simulink model "Drone_Response_v5"  (R2024b)
settings: Solver=VariableStepAuto  StartTime=0.0  StopTime=17.980265000000003  MaxStep=0.01  RelTol=1e-6  AbsTol=1e-8
model workspace (MAT data in the model file):
  Fx_gust = 1
  Fy_gust = 1
  Fz_gust = 0.5
  Ixx = 0.05
  Iyy = 0.05
  Izz = 0.1
  Kd_phi = 0.5
  Kd_psi = 0.12
  Kd_theta = 0.28
  Kd_x = 0.5
  Kd_y = 0.5
  Kd_z = 12
  Ki_phi = 0
  Ki_psi = 0
  Ki_theta = 0.28
  Ki_x = 0
  Ki_y = 0
  Ki_z = 0.1
  Kp_phi = 1
  Kp_psi = 0.012
  Kp_theta = 0.8
  Kp_x = 0.1
  Kp_y = 0.1
  Kp_z = 12
  N_phi = 100
  N_psi = 100
  N_theta = 100
  N_x = 100
  N_y = 100
  N_z = 100
  Tmax = 22.4649
  Tmin = 0
  d = 0.2
  disturbances_enabled = 0
  flight_mode = 3
  frozen_configuration.Name = "V3_conditioned_start"
  frozen_configuration.Kp = 0.753283912428
  frozen_configuration.Kd = 1.41064730788
  frozen_configuration.FeedforwardGain = 0.856563645814
  frozen_configuration.KpX = 0.1
  frozen_configuration.KdX = 0.192
  frozen_configuration.KpY = 0.1
  frozen_configuration.KdY = 0.192
  frozen_configuration.KpYaw = 0.012
  frozen_configuration.KdYaw = 0.12
  frozen_configuration.DragRate = 0
  frozen_configuration.ConditionAllFilters = 1
  frozen_configuration.Ki = 0.0024123505433
  frozen_filter_init_184 = 0.000968325935072
  frozen_filter_init_244 = -0.00996407378017
  frozen_filter_init_247 = 0.0189310533866
  frozen_filter_init_63 = 0.120731046274
  frozen_filter_init_8 = -0.00230151225217
  frozen_filter_init_92 = -0.00686694318858
  g = 9.81
  inv_m = 0.333333333333
  kf = 4e-05
  km = 1e-06
  m = 3
  mg = 29.43
  omega_hover = 399.217985567
  omega_init = 428.879353665
  phi0 = 0.0109224523708
  phi_des = 0
  phi_dot0 = -0.0602280499979
  phi_manual = 0
  pitch_pair_allocation = 2.5
  psi0 = 2.78260847334
  psi_des = 0
  psi_dot0 = 0.0811475700195
  psi_hold = 0
  psi_manual = 0
  rad_to_deg = 57.2957795131
  replay_collective_to_pair_thrust_N = 58
  replay_enabled = 1
  replay_hover_collective = 0.24829455053
  replay_hover_pair_thrust_scale_N = 51.3503013771
  response_axis_nx = -0.0174524064373
  response_axis_ny = 0
  response_axis_nz = 0.999847695156
  response_experiment_status = 'Frozen experimental replay: ascent training8.7805; reserved descent2.6653; full airborne0. NOT a general8/10 release.'
  response_manual_enable = timeseries
  response_manual_enable.Name = 'unnamed'
  response_manual_enable.DataInfo = tsdata.datametadata
  response_manual_enable.DataInfo.Interpolation = tsdata.interpolation
  response_manual_enable.DataInfo.Interpolation.Fhandle : function handle (value not decoded)
  response_manual_enable.DataInfo.Interpolation.Name = 'zoh'
  response_manual_enable.TimeInfo = tsdata.timemetadata
  response_manual_enable.TimeInfo.Length = 3
  response_manual_enable.TimeInfo.DuplicateTimes = 0
  response_manual_enable.TimeInfo.Time_ = [0; 5.880394; 17.980265]
  response_manual_enable.TimeInfo.Initialized = 1
  response_manual_enable.QualityInfo = tsdata.qualmetadata
  response_manual_enable.Data_ = [1; 0; 0]
  response_v5_status = 'Experimental controller design; general8/10 not achieved; manufacturer cap provisional'
  response_vertical_drag_rate = 0.5
  roll_motor_allocation = 1.25
  rtl_accel_ff_gain = 0.856563645814
  rtl_altitude_accel_command = timeseries
  rtl_altitude_accel_command.Name = 'unnamed'
  rtl_altitude_accel_command.DataInfo = tsdata.datametadata
  rtl_altitude_accel_command.DataInfo.Interpolation = tsdata.interpolation
  rtl_altitude_accel_command.DataInfo.Interpolation.Fhandle : function handle (value not decoded)
  rtl_altitude_accel_command.DataInfo.Interpolation.Name = 'linear'
  rtl_altitude_accel_command.TimeInfo = tsdata.timemetadata
  rtl_altitude_accel_command.TimeInfo.Length = 123
  rtl_altitude_accel_command.TimeInfo.DuplicateTimes = 0
  rtl_altitude_accel_command.TimeInfo.Time_ = [0; 5.880394; 5.980272; 6.080277; 6.180255; 6.28026; 6.380282; 6.480267; 6.58025; 6.680284; 6.780266; 6.880307; 6.980304; 7.080327; 7.180309; 7.28036; 7.380272; 7.480369; 7.580265; 7.680303; 7.780327; 7.88026; 7.980267; 8.0803; 8.180255; 8.280288; 8.380371; 8.480426; 8.580296; 8.680242; 8.780295; 8.880341; 8.980333; 9.080338; 9.18028; 9.280281; 9.38027; 9.480349; 9.580281; 9.680319; 9.780339; 9.880364; 9.980252; 10.08027; 10.180295; 10.280293; 10.380328; 10.480356; 10.580361; 10.680314; 10.780279; 10.880304; 10.980348; 11.080341; 11.180274; 11.280283; 11.380309; 11.480356; 11.580307; 11.680321; 11.780293; 11.880341; 11.980295; 12.080556; 12.180476; 12.280509; 12.380582; 12.480512; 12.580546; 12.680601; 12.780541; 12.88065; 12.98044; 13.080515; 13.1805; 13.280467; 13.380502; 13.480479; 13.580213; 13.680301; 13.78037; 13.880285; 13.980348; 14.080256; 14.180283; 14.280267; 14.380331; 14.480276; 14.580289; 14.680347; 14.780427; 14.880325; 14.980354; 15.080269; 15.180342; 15.280291; 15.380296; 15.480345; 15.58038; 15.680328; 15.780405; 15.880354; 15.980314; 16.080371; 16.180263; 16.280315; 16.38031; 16.480339; 16.580342; 16.680388; 16.780251; 16.880439; 16.980399; 17.080319; 17.180393; 17.28056; 17.380538; 17.480514; 17.580544; 17.680543; 17.780504; 17.880606; 17.980265]
  rtl_altitude_accel_command.TimeInfo.Initialized = 1
  rtl_altitude_accel_command.QualityInfo = tsdata.qualmetadata
  rtl_altitude_accel_command.Data_ = [0; 0; 0.0181679464877; 0.0999046862125; 0.199560061097; 0.298722893; 0.397746771574; 0.496650129557; 0.594934642315; 0.692368984222; 0.789256870747; 0.885816633701; 0.971697807312; 0.999798774719; 1; 1; 0.998033642769; 0.953759610653; 0.861082315445; 0.764516830444; 0.667832434177; 0.571011126041; 0.474065184593; 0.376998990774; 0.279818117619; 0.182528525591; 0.085197865963; 0.0125827109441; -2.03635991056e-05; -0.0222320128232; -0.105447649956; -0.203315362334; -0.301267236471; -0.399298965931; -0.497407704592; -0.595590174198; -0.693845033646; -0.792165696621; -0.890553176403; -0.975875973701; -0.999960243702; -1; -1; -0.995349287987; -0.938295960426; -0.841576755047; -0.744714379311; -0.649171352386; -0.554860889912; -0.46153691411; -0.368872374296; -0.276544451714; -0.184268996119; -0.0918518081307; -0.0177598670125; -5.03206729263e-06; 0; 0; 0; 0; 0; 0; 0; 0; 0; 0; 0; 0; 0; 0; 0; 0; 0; 0; 0; 0; 0; 0; 0; 0; 0; 0; 0; 0; 0; 0; 0; 0; 0; 0; 0; 0; 0; 0; -0.0749799907207; -0.574979841709; -1.07501459122; -1.5749809742; -2.07498693466; -2.5; -2.5; -2.5; -2.20005011559; -1.80034160614; -1.47325873375; -1.20559740067; -0.986563205719; -0.807322978973; -0.660650730133; -0.540626049042; -0.442403793335; -0.362028121948; -0.296255111694; -0.242431640625; -0.198386669159; -0.162343978882; -0.132850646973; -0.108713150024; -0.0889620780945; -0.0808801651001; -0.0808801651001; -0.0808801651001; -0.0808801651001]
  rtl_altitude_command = timeseries
  rtl_altitude_command.Name = 'unnamed'
  rtl_altitude_command.DataInfo = tsdata.datametadata
  rtl_altitude_command.DataInfo.Interpolation = tsdata.interpolation
  rtl_altitude_command.DataInfo.Interpolation.Fhandle : function handle (value not decoded)
  rtl_altitude_command.DataInfo.Interpolation.Name = 'linear'
  rtl_altitude_command.TimeInfo = tsdata.timemetadata
  rtl_altitude_command.TimeInfo.Length = 123
  rtl_altitude_command.TimeInfo.DuplicateTimes = 0
  rtl_altitude_command.TimeInfo.Time_ = [0; 5.880394; 5.979983; 6.07999; 6.179964; 6.279978; 6.379976; 6.479917; 6.579989; 6.679992; 6.779968; 6.879977; 6.979963; 7.080021; 7.17998; 7.280018; 7.379989; 7.479986; 7.579979; 7.679968; 7.779937; 7.879919; 7.979972; 8.079955; 8.179966; 8.279955; 8.379991; 8.479999; 8.579956; 8.679932; 8.77995; 8.879967; 8.980013; 9.079979; 9.179962; 9.279998; 9.37998; 9.48003; 9.579994; 9.68008; 9.779967; 9.879998; 9.979923; 10.079984; 10.17999; 10.279955; 10.379992; 10.479965; 10.579996; 10.67994; 10.779994; 10.87998; 10.979974; 11.079939; 11.179959; 11.279989; 11.379969; 11.479998; 11.579954; 11.679969; 11.779967; 11.880011; 11.980006; 12.080225; 12.18023; 12.280217; 12.380242; 12.480157; 12.580185; 12.680211; 12.780147; 12.880229; 12.98014; 13.080206; 13.180149; 13.280169; 13.380193; 13.480181; 13.57997; 13.679988; 13.779992; 13.879966; 13.979968; 14.079977; 14.179944; 14.279969; 14.379982; 14.479969; 14.579948; 14.680005; 14.78005; 14.879995; 14.980013; 15.079985; 15.180018; 15.280039; 15.380008; 15.480012; 15.580013; 15.680018; 15.780057; 15.880002; 15.979997; 16.079991; 16.179996; 16.280032; 16.380004; 16.480045; 16.580054; 16.680036; 16.77999; 16.879998; 16.980065; 17.080013; 17.180054; 17.280245; 17.380202; 17.480216; 17.580208; 17.68019; 17.780209; 17.880237; 17.980265]
  rtl_altitude_command.TimeInfo.Initialized = 1
  rtl_altitude_command.QualityInfo = tsdata.qualmetadata
  rtl_altitude_command.Data_ = [0.367621053576; 0.483209289175; 0.483218938112; 0.483470082283; 0.484722971916; 0.487935483456; 0.494074642658; 0.504099428654; 0.518872797489; 0.539188861847; 0.565907895565; 0.599907636642; 0.642079949379; 0.693213403225; 0.753614664078; 0.823296189308; 0.902249276638; 0.990441262722; 1.08753430843; 1.19278562069; 1.30530929565; 1.42424869537; 1.54870462418; 1.67777895927; 1.81056404114; 1.94614470005; 2.08360695839; 2.22203707695; 2.36078095436; 2.49964690208; 2.63837504387; 2.77620983124; 2.91221284866; 3.04543209076; 3.17491340637; 3.2996981144; 3.41882610321; 3.53132796288; 3.63623952866; 3.73261880875; 3.81959486008; 3.89694857597; 3.96462106705; 4.02259063721; 4.07086610794; 4.10985040665; 4.1404504776; 4.16378450394; 4.18100118637; 4.19317579269; 4.20128536224; 4.20621347427; 4.20878314972; 4.20978498459; 4.20999193192; 4.21000099182; 4.21000099182; 4.21000099182; 4.21000099182; 4.21000099182; 4.21000099182; 4.21000099182; 4.21000099182; 4.21000099182; 4.21000099182; 4.21000099182; 4.21000099182; 4.21000099182; 4.21000099182; 4.21000099182; 4.21000099182; 4.21000099182; 4.21000099182; 4.21000099182; 4.21000099182; 4.21000099182; 4.21000099182; 4.21000099182; 4.21000099182; 4.21000099182; 4.21000099182; 4.21000099182; 4.21000099182; 4.21000099182; 4.21000099182; 4.21000099182; 4.21000099182; 4.21000099182; 4.21000099182; 4.21000099182; 4.21000099182; 4.21000099182; 4.21000099182; 4.21000099182; 4.20999908447; 4.20877456665; 4.20186281204; 4.18426465988; 4.15097808838; 4.09700679779; 4.01857089996; 3.91513323784; 3.78689551353; 3.63657021523; 3.46813893318; 3.28488707542; 3.08950638771; 2.88419985771; 2.67078113556; 2.45071744919; 2.22520899773; 1.99525260925; 1.76165485382; 1.52507710457; 1.28606081009; 1.04504907131; 0.802404284477; 0.558423280716; 0.313348680735; 0.153572425246; 0.153572425246; 0.153572425246; 0.153572425246]
  rtl_altitude_filter_init = 0.354897972076
  rtl_attitude_inputs = Simulink.SimulationData.Dataset
  rtl_attitude_inputs.any.Name = ''
  rtl_attitude_inputs.any.Version = 3
  rtl_attitude_inputs.any.Storage = Simulink.SimulationData.Storage.RamDatasetStorage
  rtl_attitude_inputs.any.Storage.any.Version = 2
  rtl_attitude_inputs.any.Storage.any.Elements{1} = timeseries
  rtl_attitude_inputs.any.Storage.any.Elements{1}.Name = 'unnamed'
  rtl_attitude_inputs.any.Storage.any.Elements{1}.DataInfo = tsdata.datametadata
  rtl_attitude_inputs.any.Storage.any.Elements{1}.DataInfo.Interpolation = tsdata.interpolation
  rtl_attitude_inputs.any.Storage.any.Elements{1}.DataInfo.Interpolation.Fhandle : function handle (value not decoded)
  rtl_attitude_inputs.any.Storage.any.Elements{1}.DataInfo.Interpolation.Name = 'linear'
  rtl_attitude_inputs.any.Storage.any.Elements{1}.TimeInfo = tsdata.timemetadata
  rtl_attitude_inputs.any.Storage.any.Elements{1}.TimeInfo.Length = 181
  rtl_attitude_inputs.any.Storage.any.Elements{1}.TimeInfo.DuplicateTimes = 0
  rtl_attitude_inputs.any.Storage.any.Elements{1}.TimeInfo.Time_ = [0; 0.080274; 0.1802; 0.280234; 0.380222; 0.480249; 0.580253; 0.680152; 0.780224; 0.88031; 0.980226; 1.079987; 1.179992; 1.279971; 1.379979; 1.47997; 1.579965; 1.680013; 1.779983; 1.880027; 1.979992; 2.080025; 2.180002; 2.279959; 2.379992; 2.479963; 2.579984; 2.679956; 2.779991; 2.880052; 2.979992; 3.079983; 3.179983; 3.279973; 3.38001; 3.479962; 3.579979; 3.67989; 3.779954; 3.880051; 3.979978; 4.079962; 4.179986; 4.279998; 4.379911; 4.480031; 4.579976; 4.679978; 4.779976; 4.880011; 4.979973; 5.079962; 5.179974; 5.279962; 5.379967; 5.479959; 5.579952; 5.67998; 5.779943; 5.880155; 5.98003; 6.080038; 6.180012; 6.280028; 6.38006; 6.480004; 6.580054; 6.680046; 6.780061; 6.880107; 6.980027; 7.080069; 7.180028; 7.280073; 7.380037; 7.480075; 7.580032; 7.680054; 7.780023; 7.880064; 7.980019; 8.080031; 8.180013; 8.28005; 8.380053; 8.480122; 8.580035; 8.680023; 8.78003; 8.880101; 8.980065; 9.080052; 9.180038; 9.280062; 9.380053; 9.480077; 9.580042; 9.680127; 9.780055; 9.880099; 9.980051; 10.080031; 10.180051; 10.280051; 10.380047; 10.480059; 10.580044; 10.680028; 10.780041; 10.880067; 10.980026; 11.080039; 11.180026; 11.28004; 11.380018; 11.480049; 11.580021; 11.680058; 11.780082; 11.880129; 11.980069; 12.080272; 12.180278; 12.280307; 12.380303; 12.480207; 12.580245; 12.680299; 12.780197; 12.880404; 12.980187; 13.080253; 13.180196; 13.280216; 13.380267; 13.480231; 13.58002; 13.68007; 13.780054; 13.88009; 13.980057; 14.080025; 14.180037; 14.280028; 14.380082; 14.480019; 14.580051; 14.680069; 14.780127; 14.880083; 14.980064; 15.080032; 15.180067; 15.280099; 15.380054; 15.480087; 15.580079; 15.680088; 15.780108; 15.880123; 15.980062; 16.080038; 16.180066; 16.280082; 16.380115; 16.480093; 16.580101; 16.680095; 16.780041; 16.880161; 16.980113; 17.080083; 17.180101; 17.280292; 17.380289; 17.480263; 17.580286; 17.680277; 17.780257; 17.880352; 17.980265]
  rtl_attitude_inputs.any.Storage.any.Elements{1}.TimeInfo.Initialized = 1
  rtl_attitude_inputs.any.Storage.any.Elements{1}.QualityInfo = tsdata.qualmetadata
  rtl_attitude_inputs.any.Storage.any.Elements{1}.Data_ = [1.94907928221e-06 1.94907928221e-06 1.94907928221e-06 1.94907928221e-06 1.94907928221e-06 1.94907928221e-06 1.94907928221e-06 1.94907928221e-06 1.94907928221e-06 1.94907928221e-06 1.94907928221e-06 1.94907928221e-06 ... (181 elements, 181x1)]
  rtl_attitude_inputs.any.Storage.any.Elements{2} = timeseries
  rtl_attitude_inputs.any.Storage.any.Elements{2}.Name = 'unnamed'
  rtl_attitude_inputs.any.Storage.any.Elements{2}.DataInfo = tsdata.datametadata
  rtl_attitude_inputs.any.Storage.any.Elements{2}.DataInfo.Interpolation = tsdata.interpolation
  rtl_attitude_inputs.any.Storage.any.Elements{2}.DataInfo.Interpolation.Fhandle : function handle (value not decoded)
  rtl_attitude_inputs.any.Storage.any.Elements{2}.DataInfo.Interpolation.Name = 'linear'
  rtl_attitude_inputs.any.Storage.any.Elements{2}.TimeInfo = tsdata.timemetadata
  rtl_attitude_inputs.any.Storage.any.Elements{2}.TimeInfo.Length = 181
  rtl_attitude_inputs.any.Storage.any.Elements{2}.TimeInfo.DuplicateTimes = 0
  rtl_attitude_inputs.any.Storage.any.Elements{2}.TimeInfo.Time_ = [0; 0.080274; 0.1802; 0.280234; 0.380222; 0.480249; 0.580253; 0.680152; 0.780224; 0.88031; 0.980226; 1.079987; 1.179992; 1.279971; 1.379979; 1.47997; 1.579965; 1.680013; 1.779983; 1.880027; 1.979992; 2.080025; 2.180002; 2.279959; 2.379992; 2.479963; 2.579984; 2.679956; 2.779991; 2.880052; 2.979992; 3.079983; 3.179983; 3.279973; 3.38001; 3.479962; 3.579979; 3.67989; 3.779954; 3.880051; 3.979978; 4.079962; 4.179986; 4.279998; 4.379911; 4.480031; 4.579976; 4.679978; 4.779976; 4.880011; 4.979973; 5.079962; 5.179974; 5.279962; 5.379967; 5.479959; 5.579952; 5.67998; 5.779943; 5.880155; 5.98003; 6.080038; 6.180012; 6.280028; 6.38006; 6.480004; 6.580054; 6.680046; 6.780061; 6.880107; 6.980027; 7.080069; 7.180028; 7.280073; 7.380037; 7.480075; 7.580032; 7.680054; 7.780023; 7.880064; 7.980019; 8.080031; 8.180013; 8.28005; 8.380053; 8.480122; 8.580035; 8.680023; 8.78003; 8.880101; 8.980065; 9.080052; 9.180038; 9.280062; 9.380053; 9.480077; 9.580042; 9.680127; 9.780055; 9.880099; 9.980051; 10.080031; 10.180051; 10.280051; 10.380047; 10.480059; 10.580044; 10.680028; 10.780041; 10.880067; 10.980026; 11.080039; 11.180026; 11.28004; 11.380018; 11.480049; 11.580021; 11.680058; 11.780082; 11.880129; 11.980069; 12.080272; 12.180278; 12.280307; 12.380303; 12.480207; 12.580245; 12.680299; 12.780197; 12.880404; 12.980187; 13.080253; 13.180196; 13.280216; 13.380267; 13.480231; 13.58002; 13.68007; 13.780054; 13.88009; 13.980057; 14.080025; 14.180037; 14.280028; 14.380082; 14.480019; 14.580051; 14.680069; 14.780127; 14.880083; 14.980064; 15.080032; 15.180067; 15.280099; 15.380054; 15.480087; 15.580079; 15.680088; 15.780108; 15.880123; 15.980062; 16.080038; 16.180066; 16.280082; 16.380115; 16.480093; 16.580101; 16.680095; 16.780041; 16.880161; 16.980113; 17.080083; 17.180101; 17.280292; 17.380289; 17.480263; 17.580286; 17.680277; 17.780257; 17.880352; 17.980265]
  rtl_attitude_inputs.any.Storage.any.Elements{2}.TimeInfo.Initialized = 1
  rtl_attitude_inputs.any.Storage.any.Elements{2}.QualityInfo = tsdata.qualmetadata
  rtl_attitude_inputs.any.Storage.any.Elements{2}.Data_ = [4.06449793757e-06 4.06449793757e-06 4.06449793757e-06 4.06449793757e-06 4.06449793757e-06 4.06449793757e-06 4.06449793757e-06 4.06449793757e-06 4.06449793757e-06 4.06449793757e-06 4.06449793757e-06 4.06449793757e-06 ... (181 elements, 181x1)]
  rtl_attitude_inputs.any.Storage.any.Elements{3} = timeseries
  rtl_attitude_inputs.any.Storage.any.Elements{3}.Name = 'unnamed'
  rtl_attitude_inputs.any.Storage.any.Elements{3}.DataInfo = tsdata.datametadata
  rtl_attitude_inputs.any.Storage.any.Elements{3}.DataInfo.Interpolation = tsdata.interpolation
  rtl_attitude_inputs.any.Storage.any.Elements{3}.DataInfo.Interpolation.Fhandle : function handle (value not decoded)
  rtl_attitude_inputs.any.Storage.any.Elements{3}.DataInfo.Interpolation.Name = 'linear'
  rtl_attitude_inputs.any.Storage.any.Elements{3}.TimeInfo = tsdata.timemetadata
  rtl_attitude_inputs.any.Storage.any.Elements{3}.TimeInfo.Length = 181
  rtl_attitude_inputs.any.Storage.any.Elements{3}.TimeInfo.DuplicateTimes = 0
  rtl_attitude_inputs.any.Storage.any.Elements{3}.TimeInfo.Time_ = [0; 0.080274; 0.1802; 0.280234; 0.380222; 0.480249; 0.580253; 0.680152; 0.780224; 0.88031; 0.980226; 1.079987; 1.179992; 1.279971; 1.379979; 1.47997; 1.579965; 1.680013; 1.779983; 1.880027; 1.979992; 2.080025; 2.180002; 2.279959; 2.379992; 2.479963; 2.579984; 2.679956; 2.779991; 2.880052; 2.979992; 3.079983; 3.179983; 3.279973; 3.38001; 3.479962; 3.579979; 3.67989; 3.779954; 3.880051; 3.979978; 4.079962; 4.179986; 4.279998; 4.379911; 4.480031; 4.579976; 4.679978; 4.779976; 4.880011; 4.979973; 5.079962; 5.179974; 5.279962; 5.379967; 5.479959; 5.579952; 5.67998; 5.779943; 5.880155; 5.98003; 6.080038; 6.180012; 6.280028; 6.38006; 6.480004; 6.580054; 6.680046; 6.780061; 6.880107; 6.980027; 7.080069; 7.180028; 7.280073; 7.380037; 7.480075; 7.580032; 7.680054; 7.780023; 7.880064; 7.980019; 8.080031; 8.180013; 8.28005; 8.380053; 8.480122; 8.580035; 8.680023; 8.78003; 8.880101; 8.980065; 9.080052; 9.180038; 9.280062; 9.380053; 9.480077; 9.580042; 9.680127; 9.780055; 9.880099; 9.980051; 10.080031; 10.180051; 10.280051; 10.380047; 10.480059; 10.580044; 10.680028; 10.780041; 10.880067; 10.980026; 11.080039; 11.180026; 11.28004; 11.380018; 11.480049; 11.580021; 11.680058; 11.780082; 11.880129; 11.980069; 12.080272; 12.180278; 12.280307; 12.380303; 12.480207; 12.580245; 12.680299; 12.780197; 12.880404; 12.980187; 13.080253; 13.180196; 13.280216; 13.380267; 13.480231; 13.58002; 13.68007; 13.780054; 13.88009; 13.980057; 14.080025; 14.180037; 14.280028; 14.380082; 14.480019; 14.580051; 14.680069; 14.780127; 14.880083; 14.980064; 15.080032; 15.180067; 15.280099; 15.380054; 15.480087; 15.580079; 15.680088; 15.780108; 15.880123; 15.980062; 16.080038; 16.180066; 16.280082; 16.380115; 16.480093; 16.580101; 16.680095; 16.780041; 16.880161; 16.980113; 17.080083; 17.180101; 17.280292; 17.380289; 17.480263; 17.580286; 17.680277; 17.780257; 17.880352; 17.980265]
  rtl_attitude_inputs.any.Storage.any.Elements{3}.TimeInfo.Initialized = 1
  rtl_attitude_inputs.any.Storage.any.Elements{3}.QualityInfo = tsdata.qualmetadata
  rtl_attitude_inputs.any.Storage.any.Elements{3}.Data_ = [2.71005829161 2.71005829161 2.71005829161 2.71005829161 2.71005829161 2.71005829161 2.71005829161 2.71005829161 2.71005829161 2.71005829161 2.71005829161 2.71005829161 ... (181 elements, 181x1)]
  rtl_attitude_inputs.any.Storage.any.Elements{4} = timeseries
  rtl_attitude_inputs.any.Storage.any.Elements{4}.Name = 'unnamed'
  rtl_attitude_inputs.any.Storage.any.Elements{4}.DataInfo = tsdata.datametadata
  rtl_attitude_inputs.any.Storage.any.Elements{4}.DataInfo.Interpolation = tsdata.interpolation
  rtl_attitude_inputs.any.Storage.any.Elements{4}.DataInfo.Interpolation.Fhandle : function handle (value not decoded)
  rtl_attitude_inputs.any.Storage.any.Elements{4}.DataInfo.Interpolation.Name = 'linear'
  rtl_attitude_inputs.any.Storage.any.Elements{4}.TimeInfo = tsdata.timemetadata
  rtl_attitude_inputs.any.Storage.any.Elements{4}.TimeInfo.Length = 181
  rtl_attitude_inputs.any.Storage.any.Elements{4}.TimeInfo.DuplicateTimes = 0
  rtl_attitude_inputs.any.Storage.any.Elements{4}.TimeInfo.Time_ = [0; 0.080227; 0.180111; 0.280186; 0.380174; 0.480171; 0.580174; 0.680103; 0.780135; 0.880162; 0.980132; 1.07994; 1.179943; 1.279883; 1.379885; 1.479879; 1.579917; 1.679925; 1.779889; 1.879916; 1.979912; 2.079935; 2.179952; 2.27988; 2.379914; 2.479913; 2.579884; 2.679905; 2.779893; 2.879917; 2.979944; 3.079936; 3.179931; 3.279898; 3.379921; 3.47987; 3.579932; 3.679842; 3.779905; 3.879944; 3.97993; 4.079914; 4.179938; 4.27995; 4.379861; 4.479943; 4.579887; 4.679927; 4.779875; 4.879885; 4.979885; 5.079914; 5.179924; 5.279885; 5.37992; 5.479911; 5.579905; 5.679892; 5.779864; 5.880014; 5.979983; 6.07999; 6.179964; 6.279978; 6.379976; 6.479917; 6.579989; 6.679992; 6.779968; 6.879977; 6.979963; 7.080021; 7.17998; 7.280018; 7.379989; 7.479986; 7.579979; 7.679968; 7.779937; 7.879919; 7.979972; 8.079955; 8.179966; 8.279955; 8.379991; 8.479999; 8.579956; 8.679932; 8.77995; 8.879967; 8.980013; 9.079979; 9.179962; 9.279998; 9.37998; 9.48003; 9.579994; 9.68008; 9.779967; 9.879998; 9.979923; 10.079984; 10.17999; 10.279955; 10.379992; 10.479965; 10.579996; 10.67994; 10.779994; 10.87998; 10.979974; 11.079939; 11.179959; 11.279989; 11.379969; 11.479998; 11.579954; 11.679969; 11.779967; 11.880011; 11.980006; 12.080225; 12.18023; 12.280217; 12.380242; 12.480157; 12.580185; 12.680211; 12.780147; 12.880229; 12.98014; 13.080206; 13.180149; 13.280169; 13.380193; 13.480181; 13.57997; 13.679988; 13.779992; 13.879966; 13.979968; 14.079977; 14.179944; 14.279969; 14.379982; 14.479969; 14.579948; 14.680005; 14.78005; 14.879995; 14.980013; 15.079985; 15.180018; 15.280039; 15.380008; 15.480012; 15.580013; 15.680018; 15.780057; 15.880002; 15.979997; 16.079991; 16.179996; 16.280032; 16.380004; 16.480045; 16.580054; 16.680036; 16.77999; 16.879998; 16.980065; 17.080013; 17.180054; 17.280245; 17.380202; 17.480216; 17.580208; 17.68019; 17.780209; 17.880237; 17.980265]
  rtl_attitude_inputs.any.Storage.any.Elements{4}.TimeInfo.Initialized = 1
  rtl_attitude_inputs.any.Storage.any.Elements{4}.QualityInfo = tsdata.qualmetadata
  rtl_attitude_inputs.any.Storage.any.Elements{4}.Data_ = [0.2475470274 0.247529372573 0.247571662068 0.247633695602 0.247520431876 0.247513592243 0.247479513288 0.250810205936 0.250822991133 0.251647055149 0.255733072758 0.258190184832 ... (181 elements, 181x1)]
  rtl_drag_rate = 1
  rtl_east_target = timeseries
  rtl_east_target.Name = 'unnamed'
  rtl_east_target.DataInfo = tsdata.datametadata
  rtl_east_target.DataInfo.Interpolation = tsdata.interpolation
  rtl_east_target.DataInfo.Interpolation.Fhandle : function handle (value not decoded)
  rtl_east_target.DataInfo.Interpolation.Name = 'linear'
  rtl_east_target.TimeInfo = tsdata.timemetadata
  rtl_east_target.TimeInfo.Length = 123
  rtl_east_target.TimeInfo.DuplicateTimes = 0
  rtl_east_target.TimeInfo.Time_ = [0; 5.880394; 5.980267; 6.080272; 6.180251; 6.280255; 6.380278; 6.480263; 6.580245; 6.680279; 6.780261; 6.880302; 6.980299; 7.080322; 7.180304; 7.280356; 7.380267; 7.480364; 7.580261; 7.680298; 7.780322; 7.880255; 7.980263; 8.080296; 8.18025; 8.280283; 8.380367; 8.48042; 8.580291; 8.680238; 8.780291; 8.880337; 8.980328; 9.080333; 9.180275; 9.280264; 9.380265; 9.480345; 9.580274; 9.680314; 9.780322; 9.880359; 9.980248; 10.080265; 10.180291; 10.280288; 10.380323; 10.480351; 10.580357; 10.68031; 10.780274; 10.880299; 10.980343; 11.080336; 11.18027; 11.280279; 11.380275; 11.480351; 11.580303; 11.680317; 11.780288; 11.880337; 11.98029; 12.080551; 12.180466; 12.280505; 12.380577; 12.480507; 12.580542; 12.680596; 12.780537; 12.880646; 12.980435; 13.080511; 13.180495; 13.280449; 13.380497; 13.48047; 13.580208; 13.680296; 13.780366; 13.880277; 13.980322; 14.080251; 14.180278; 14.280263; 14.380326; 14.480271; 14.580284; 14.680342; 14.780422; 14.880321; 14.980349; 15.080265; 15.180337; 15.280287; 15.380292; 15.48034; 15.580375; 15.680324; 15.780401; 15.88035; 15.980309; 16.08034; 16.180258; 16.280311; 16.380305; 16.480334; 16.580337; 16.680352; 16.780246; 16.880434; 16.980394; 17.080315; 17.180388; 17.280544; 17.380533; 17.480509; 17.58054; 17.680538; 17.7805; 17.880601; 17.980265]
  rtl_east_target.TimeInfo.Initialized = 1
  rtl_east_target.QualityInfo = tsdata.qualmetadata
  rtl_east_target.Data_ = [0; 0.248018814352; 0.248018823665; 0.248019067672; 0.248020287704; 0.248023413223; 0.248029388588; 0.248039145124; 0.248053522882; 0.24807329486; 0.248099297386; 0.248132385415; 0.248173428801; 0.248223191228; 0.248281974447; 0.248349789631; 0.248426627469; 0.248512456295; 0.248606948283; 0.248709380728; 0.248818889361; 0.248934643444; 0.249055763808; 0.249181380597; 0.249310609054; 0.249442556974; 0.249576335874; 0.249711057272; 0.249846084145; 0.249981230226; 0.250116242197; 0.250250384313; 0.250382743877; 0.250512393293; 0.250638406825; 0.250759847563; 0.25087632994; 0.251004878533; 0.25121394555; 0.251599053022; 0.252257388186; 0.253287786719; 0.254789102924; 0.256860426728; 0.259593957205; 0.263035087947; 0.267160802715; 0.271908525391; 0.277184148886; 0.282897299257; 0.288973314789; 0.295345921171; 0.301952984285; 0.308729320866; 0.315602529895; 0.322515800696; 0.329449839991; 0.336387127739; 0.343267537755; 0.350006468695; 0.356516786021; 0.362709790569; 0.36849550913; 0.373783595961; 0.378482692045; 0.38251579563; 0.385851591927; 0.388496592742; 0.390504479509; 0.391959562999; 0.392949804765; 0.393563933772; 0.393890813094; 0.394023783606; 0.394056178731; 0.39405874173; 0.394058764082; 0.394058764082; 0.394058764082; 0.394058764082; 0.394058764082; 0.394058764082; 0.394058764082; 0.394058764082; 0.394058764082; 0.394058764082; 0.394058764082; 0.394058764082; 0.394058764082; 0.394058764082; 0.394058764082; 0.394058764082; 0.394058764082; 0.394058764082; 0.430912442607; 0.428267322582; 0.425051026147; 0.421733401817; 0.418574698371; 0.415684960884; 0.413093470138; 0.410792537135; 0.408759869736; 0.406968586248; 0.40539199869; 0.404005400938; 0.402786545557; 0.401715271276; 0.400773637098; 0.399945788187; 0.399218119782; 0.398578889769; 0.398017488521; 0.397524453801; 0.397091485661; 0.396711289984; 0.396377474171; 0.396084465188; 0.395827353102; 0.395601876181; 0.395404182476; 0.395231179994; 0.395231179994]
  rtl_north_target = timeseries
  rtl_north_target.Name = 'unnamed'
  rtl_north_target.DataInfo = tsdata.datametadata
  rtl_north_target.DataInfo.Interpolation = tsdata.interpolation
  rtl_north_target.DataInfo.Interpolation.Fhandle : function handle (value not decoded)
  rtl_north_target.DataInfo.Interpolation.Name = 'linear'
  rtl_north_target.TimeInfo = tsdata.timemetadata
  rtl_north_target.TimeInfo.Length = 123
  rtl_north_target.TimeInfo.DuplicateTimes = 0
  rtl_north_target.TimeInfo.Time_ = [0; 5.880394; 5.980263; 6.080268; 6.180246; 6.280251; 6.380273; 6.480258; 6.58024; 6.680275; 6.780257; 6.880298; 6.980295; 7.080318; 7.1803; 7.280351; 7.380263; 7.48036; 7.580256; 7.680294; 7.780318; 7.880247; 7.980258; 8.080291; 8.180246; 8.280279; 8.380362; 8.480403; 8.580286; 8.680233; 8.780286; 8.880332; 8.980323; 9.080317; 9.18027; 9.280241; 9.380261; 9.48034; 9.580269; 9.68031; 9.780317; 9.880355; 9.980243; 10.080261; 10.180286; 10.280284; 10.380319; 10.480327; 10.580352; 10.680305; 10.78027; 10.880295; 10.980339; 11.080332; 11.180265; 11.280274; 11.38027; 11.480347; 11.580298; 11.680312; 11.780284; 11.880332; 11.980286; 12.080547; 12.180461; 12.2805; 12.380566; 12.480503; 12.580537; 12.680592; 12.780532; 12.880641; 12.980431; 13.080506; 13.18049; 13.280445; 13.380493; 13.480465; 13.580204; 13.680292; 13.780361; 13.880273; 13.980318; 14.080247; 14.180274; 14.280258; 14.380322; 14.480266; 14.58028; 14.680338; 14.780417; 14.880316; 14.980344; 15.080248; 15.180333; 15.280282; 15.380287; 15.480336; 15.580371; 15.680319; 15.780396; 15.880345; 15.980305; 16.080336; 16.180254; 16.280306; 16.3803; 16.48033; 16.580333; 16.680348; 16.780242; 16.880429; 16.98039; 17.08031; 17.180383; 17.280526; 17.380529; 17.480505; 17.580535; 17.680534; 17.78049; 17.880596; 17.980265]
  rtl_north_target.TimeInfo.Initialized = 1
  rtl_north_target.QualityInfo = tsdata.qualmetadata
  rtl_north_target.Data_ = [0 0.841359426902 0.8413595163 0.841362228312 0.841375728764 0.841410388865 0.841476579823 0.841584672846 0.841743966259 0.841963043131 0.842251171984 0.842617770352 ... (123 elements, 123x1)]
  seed_phi = 104
  seed_psi = 106
  seed_theta = 105
  seed_x = 101
  seed_y = 102
  seed_z = 103
  sensor_noise_enabled = 0
  sensor_noise_tau_attitude = 0.1
  sensor_noise_tau_position = 0.2
  sensor_sample_time = 0.02
  sigma_phi = 0.000349065850399
  sigma_psi = 0.000872664625997
  sigma_theta = 0.000349065850399
  sigma_x = 0.002
  sigma_y = 0.002
  sigma_z = 0.001
  t_Fx_end = 11
  t_Fx_start = 10
  t_Fy_end = 16
  t_Fy_start = 15
  t_Fz_end = 21
  t_Fz_start = 20
  t_pitch_end = 30.5
  t_pitch_start = 30
  t_roll_end = 25.5
  t_roll_start = 25
  t_step_xy = 1
  t_step_yaw = 1
  t_step_z = 0
  t_stop = 17.980265
  t_yaw_end = 35.5
  t_yaw_start = 35
  tau_m = 0.02
  tau_pitch_gust = 0.01
  tau_roll_gust = 0.01
  tau_yaw_gust = 0.002
  theta0 = 0.0291618371461
  theta_des = 0.174532925199
  theta_dot0 = 0.0296232047334
  theta_manual = 0
  tilt_max = 0.1745
  visual_arm_length = 0.35
  visual_demo_disturbances = 1
  visual_demo_sensor_noise = 0
  visual_demo_stop_time = 60
  visual_demo_yaw = 0.523598775598
  visual_frame_rate = 30
  visual_playback_speed = 4
  visual_record_video = 0
  visual_trail_length = inf
  vx0 = 0.0296084290651
  vy0 = 0.0198878378966
  vz0 = 0.0507991741846
  x0 = 0
  x_des = 4
  x_hold = 0
  x_manual = 0
  y0 = 0
  y_des = 2
  y_hold = 0
  y_manual = 0
  yaw_motor_allocation = 10
  z0 = 0.367621053576
  z_des = 1
  z_hold = 1
  z_manual = 1
libraries: slpidlib x6
(part 1 of 2)
settings Model: Creator=shiyu  LastModifiedBy=shiyu
settings DataIOCC: ExternalInput=rtl_attitude_inputs  LoadExternalInput=on

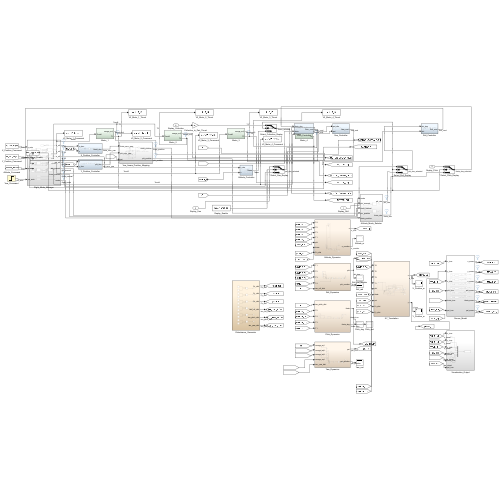
[thumbnail: Simulink's stored preview of the top-level diagram]
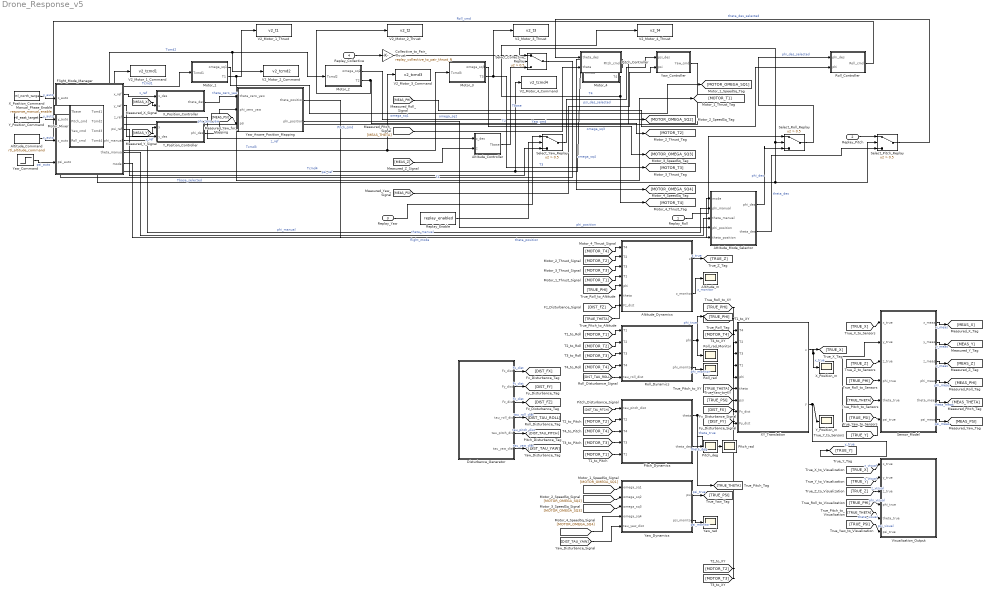
== system Drone_Response_v5 ==
  Replay_Roll : Inport
  Replay_Pitch : Inport  Port=2
  Replay_Yaw : Inport  Port=3
  Replay_Collective : Inport  Port=4
  Altitude_Command : FromWorkspace  VariableName=rtl_altitude_command
  Altitude_Controller : Subsystem  Description=Altitude error -> PID -> pair thrust correction + pair hover feed-forward. Tbase is thrust per motor pair (N).
  Altitude_Dynamics : Subsystem  Description=Inputs in unchanged port order: T4,T2,T3,T1 (N), phi,theta (rad). Both outputs are altitude (m); z_monitor duplicates z.
  Altitude_m : Scope
  Attitude_Mode_Selector : Subsystem
  Collective_to_Pair_Thrust : Gain  Gain=replay_collective_to_pair_thrust_N
  Disturbance_Generator : Subsystem  Description=Six switchable finite pulses. Outputs are world-frame forces Fx/Fy/Fz (N) and roll/pitch/yaw disturbance torques (N*m). Set disturbances_enabled=0 or 1 in Drone_parameters.m.
  Flight_Mode_Manager : Subsystem
  Manual_Phase_Enable : FromWorkspace  VariableName=response_manual_enable  Interpolate=off  OutputAfterFinalValue=Holding final value
  Motor_1 : Subsystem  Description=Motor 1: command Tcmd1 (N); output 1 omega_sq1 ((rad/s)^2), output 2 T1 (N). Rotor-speed lag and initialization preserved.
  Motor_2 : Subsystem  Description=Motor 2: command Tcmd2 (N); output 1 omega_sq2 ((rad/s)^2), output 2 T2 (N).
  Motor_3 : Subsystem  Description=Motor 3: command Tcmd3 (N); output 1 omega_sq3 ((rad/s)^2), output 2 T3 (N).
  Motor_4 : Subsystem  Description=Motor 4: command Tcmd4 (N); output 1 omega_sq4 ((rad/s)^2), output 2 T4 (N). Former Psi output was speed squared, not yaw.
  Motor_Mixer : Subsystem  Description=Input order: Tbase, Pitch_cmd, Yaw_cmd, Roll_cmd. Outputs Tcmd1..4 (N). Existing M1/M2 pair uses Tbase + Pitch_cmd; M3/M4 uses Tbase - Pitch_cmd. Do not change signs during cosmetic cleanup.
  Pitch_Controller : Subsystem  Description=Pitch angle error (rad) -> PID -> pitch pair thrust correction (N). Existing mixer sign and scaling preserved.
  Pitch_Dynamics : Subsystem  Description=Inputs: disturbance torque (N m), T2,T4,T3,T1 (N). Outputs: theta (rad), theta_deg (deg). Independent Euler-angle double integrator.
  Pitch_deg : Scope
  Pitch_rad : Scope
  Replay_Enable : Constant  Value=replay_enabled
  Roll_Controller : Subsystem  Description=Roll angle error (rad) -> PID -> per-motor differential thrust correction (N).
  Roll_Dynamics : Subsystem  Description=Inputs T1,T2,T3,T4 (N). Both outputs are roll angle (rad); phi_monitor duplicates phi. Independent Euler-angle double integrator.
  Roll_rad : Scope
  Roll_rad_Monitor : Scope
  Select_Collective_Replay : Switch  Criteria=u2 > Threshold  Threshold=0.5  SaturateOnIntegerOverflow=off  InputSameDT=off
  Select_Pitch_Replay : Switch  Criteria=u2 > Threshold  Threshold=0.5  SaturateOnIntegerOverflow=off  InputSameDT=off
  Select_Roll_Replay : Switch  Criteria=u2 > Threshold  Threshold=0.5  SaturateOnIntegerOverflow=off  InputSameDT=off
  Select_Yaw_Replay : Switch  Criteria=u2 > Threshold  Threshold=0.5  SaturateOnIntegerOverflow=off  InputSameDT=off
  Sensor_Model : Subsystem
  V2_Motor_1_Command : ToWorkspace  VariableName=v2_tcmd1  SaveFormat=Timeseries  SampleTime=-1
  V2_Motor_1_Thrust : ToWorkspace  VariableName=v2_t1  SaveFormat=Timeseries  SampleTime=-1
  V2_Motor_2_Command : ToWorkspace  VariableName=v2_tcmd2  SaveFormat=Timeseries  SampleTime=-1
  V2_Motor_2_Thrust : ToWorkspace  VariableName=v2_t2  SaveFormat=Timeseries  SampleTime=-1
  V2_Motor_3_Command : ToWorkspace  VariableName=v2_tcmd3  SaveFormat=Timeseries  SampleTime=-1
  V2_Motor_3_Thrust : ToWorkspace  VariableName=v2_t3  SaveFormat=Timeseries  SampleTime=-1
  V2_Motor_4_Command : ToWorkspace  VariableName=v2_tcmd4  SaveFormat=Timeseries  SampleTime=-1
  V2_Motor_4_Thrust : ToWorkspace  VariableName=v2_t4  SaveFormat=Timeseries  SampleTime=-1
  Visualization_Output : Subsystem
  XY_Translation : Subsystem  Description=Inputs: T4,T2,T3,T1 (N), phi,theta,psi (rad). Outputs x,y (m). Implements the ZYX body-z thrust direction: Fx/T = cos(psi)*sin(theta)*cos(phi) + sin(psi)*sin(phi); Fy/T = sin(psi)*sin(theta)*cos(phi) - cos(psi)*sin(phi). Corrected and validated 2026-09-03.
  X_Position_Command : FromWorkspace  VariableName=rtl_north_target
  X_Position_Controller : Subsystem  Description=x_des - x (m) -> existing PD -> pitch command limit (rad).
  X_Position_m : Scope
  Y_Position_Command : FromWorkspace  VariableName=rtl_east_target
  Y_Position_Controller : Subsystem  Description=Input order preserved: port 1 is actual y; port 2 is y_des. Error y_des - y, followed by existing negative roll-command sign.
  Y_Position_m : Scope
  Yaw_Aware_Position_Mapping : Subsystem
  Yaw_Command : Step  Time=t_step_yaw  After=psi_des  SampleTime=0
  Yaw_Controller : Subsystem  Description=Yaw angle error (rad) -> PID -> per-motor differential thrust correction (N).
  Yaw_Dynamics : Subsystem  Description=Inputs omega_sq1..4 ((rad/s)^2); reaction-torque coefficients are applied inside. Both outputs are yaw angle (rad); psi_monitor duplicates psi.
  Yaw_rad : Scope
  wires:
  Altitude_Dynamics/2(z_monitor) -> Altitude_m/1  "z_monitor"
  Roll_Dynamics/2(phi_monitor) -> Roll_rad/1  "phi_monitor"
  Yaw_Dynamics/2(psi_monitor) -> Yaw_rad/1  "psi_monitor"
  Pitch_Dynamics/2(theta_deg) -> Pitch_deg/1  "theta_deg"
  Flight_Mode_Manager/2(y_ref) -> Y_Position_Controller/2(y_des)  "y_ref"
  Flight_Mode_Manager/1(x_ref) -> X_Position_Controller/1(x_des)  "x_ref"
  Sensor_Model/6(psi_meas) -> [MEAS_PSI]  "psi_meas"
  Sensor_Model/5(theta_meas) -> [MEAS_THETA]  "theta_meas"
  Sensor_Model/4(phi_meas) -> [MEAS_PHI]  "phi_meas"
  Sensor_Model/3(z_meas) -> [MEAS_Z]  "z_meas"
  Sensor_Model/2(y_meas) -> [MEAS_Y]  "y_meas"
  Sensor_Model/1(x_meas) -> [MEAS_X]  "x_meas"
  XY_Translation/1(x) -> [TRUE_X], X_Position_m/1  "x_true"
  Yaw_Dynamics/1(psi) -> [TRUE_PSI]  "psi_true"
  Disturbance_Generator/1(Fx_dist) -> [DIST_FX]  "Fx_dist"
  Disturbance_Generator/2(Fy_dist) -> [DIST_FY]  "Fy_dist"
  Disturbance_Generator/3(Fz_dist) -> [DIST_FZ]  "Fz_dist"
  Disturbance_Generator/4(tau_roll_dist) -> [DIST_TAU_ROLL]  "tau_roll_dist"
  Disturbance_Generator/5(tau_pitch_dist) -> [DIST_TAU_PITCH]  "tau_pitch_dist"
  Disturbance_Generator/6(tau_yaw_dist) -> [DIST_TAU_YAW]  "tau_yaw_dist"
  X_Position_Controller/1(theta_des) -> Yaw_Aware_Position_Mapping/1(theta_zero_yaw)  "theta_zero_yaw"
  Y_Position_Controller/1(phi_des) -> Yaw_Aware_Position_Mapping/2(phi_zero_yaw)  "phi_zero_yaw"
  Altitude_Dynamics/1(z) -> [TRUE_Z]  "z_true"
  Yaw_Command/1 -> Flight_Mode_Manager/4(psi_auto)  "psi_auto"
  [MEAS_X] -> X_Position_Controller/2(x)
  [MEAS_Y] -> Y_Position_Controller/1(y)
  [MOTOR_T1] -> Altitude_Dynamics/4(T1)
  [MOTOR_T2] -> Altitude_Dynamics/2(T2)
  [MOTOR_T3] -> Altitude_Dynamics/3(T3)
  [MOTOR_T4] -> Altitude_Dynamics/1(T4)
  [MOTOR_OMEGA_SQ1] -> Yaw_Dynamics/1(omega_sq1)
  [MOTOR_OMEGA_SQ2] -> Yaw_Dynamics/2(omega_sq2)
  [MOTOR_OMEGA_SQ3] -> Yaw_Dynamics/3(omega_sq3)
  [MEAS_PSI] -> Yaw_Aware_Position_Mapping/3(psi)
  [MOTOR_T4] -> XY_Translation/1(T4)
  [MOTOR_T4] -> Pitch_Dynamics/3(T4)
  [MOTOR_T4] -> Roll_Dynamics/4(T4)
  [MOTOR_T3] -> Pitch_Dynamics/4(T3)
  [MOTOR_T3] -> Roll_Dynamics/3(T3)
  [MOTOR_T2] -> Pitch_Dynamics/2(T2)
  [MOTOR_T2] -> Roll_Dynamics/2(T2)
  [MOTOR_T1] -> Pitch_Dynamics/5(T1)
  [MOTOR_T1] -> Roll_Dynamics/1(T1)
  [TRUE_X] -> Sensor_Model/1(x_true)
  [TRUE_Z] -> Sensor_Model/3(z_true)
  [TRUE_PHI] -> Sensor_Model/4(phi_true)
  [TRUE_THETA] -> Sensor_Model/5(theta_true)
  [TRUE_PSI] -> Sensor_Model/6(psi_true)
  [TRUE_PHI] -> Altitude_Dynamics/5(phi)
  [TRUE_THETA] -> XY_Translation/6(theta)
  [TRUE_PSI] -> XY_Translation/7(psi)
  [DIST_FX] -> XY_Translation/8(Fx_dist)
  [DIST_FY] -> XY_Translation/9(Fy_dist)
  [DIST_FZ] -> Altitude_Dynamics/7(Fz_dist)
  [DIST_TAU_ROLL] -> Roll_Dynamics/5(tau_roll_dist)
  [DIST_TAU_PITCH] -> Pitch_Dynamics/1(tau_pitch_dist)
  [TRUE_PSI] -> Visualization_Output/6(psi_true)  "psi_visual"
  [TRUE_THETA] -> Visualization_Output/5(theta_true)  "theta_visual"
  [TRUE_PHI] -> Visualization_Output/4(phi_true)  "phi_visual"
  [TRUE_Z] -> Visualization_Output/3(z_true)  "z_visual"
  [TRUE_Y] -> Visualization_Output/2(y_true)  "y_visual"
  [TRUE_X] -> Visualization_Output/1(x_true)  "x_visual"
  Altitude_Controller/1(Tbase) -> Select_Collective_Replay/3  "Tbase"
  Collective_to_Pair_Thrust/1 -> Select_Collective_Replay/1
  Replay_Collective/1 -> Collective_to_Pair_Thrust/1
  Select_Yaw_Replay/1 -> Yaw_Controller/1(psi_des)  "psi_des_selected"
  Replay_Yaw/1 -> Select_Yaw_Replay/1
  Flight_Mode_Manager/4(psi_ref) -> Select_Yaw_Replay/3  "psi_ref"
  Select_Pitch_Replay/1 -> Pitch_Controller/1(theta_des)  "theta_des_selected"
  Replay_Pitch/1 -> Select_Pitch_Replay/1
  Attitude_Mode_Selector/2(theta_des) -> Select_Pitch_Replay/3  "theta_des"
  Select_Roll_Replay/1 -> Roll_Controller/1(phi_des)  "phi_des_selected"
  Replay_Enable/1 -> Select_Yaw_Replay/2
  Replay_Roll/1 -> Select_Roll_Replay/1
  Attitude_Mode_Selector/1(phi_des) -> Select_Roll_Replay/3  "phi_des"
  [MEAS_PSI] -> Yaw_Controller/2(psi)
  [MEAS_THETA] -> Pitch_Controller/2(theta)
  [MEAS_PHI] -> Roll_Controller/2(phi)
  [MEAS_Z] -> Altitude_Controller/2(z)
  Flight_Mode_Manager/3(z_ref) -> Altitude_Controller/1(z_des)  "z_ref"
  Flight_Mode_Manager/7(mode) -> Attitude_Mode_Selector/1(mode)  "flight_mode"
  Flight_Mode_Manager/5(phi_manual) -> Attitude_Mode_Selector/2(phi_manual)  "phi_manual"
  Flight_Mode_Manager/6(theta_manual) -> Attitude_Mode_Selector/3(theta_manual)  "theta_manual"
  Yaw_Aware_Position_Mapping/2(phi_position) -> Attitude_Mode_Selector/4(phi_position)  "phi_position"
  Yaw_Aware_Position_Mapping/1(theta_position) -> Attitude_Mode_Selector/5(theta_position)  "theta_position"
  Altitude_Command/1 -> Flight_Mode_Manager/3(z_auto)  "z_auto"
  X_Position_Command/1 -> Flight_Mode_Manager/1(x_auto)  "x_auto"
  Y_Position_Command/1 -> Flight_Mode_Manager/2(y_auto)  "y_auto"
  [DIST_TAU_YAW] -> Yaw_Dynamics/5(tau_yaw_dist)
  [TRUE_THETA] -> Altitude_Dynamics/6(theta)
  [TRUE_PHI] -> XY_Translation/5(phi)
  [TRUE_Y] -> Sensor_Model/2(y_true)
  [MOTOR_T1] -> XY_Translation/4(T1)
  [MOTOR_T2] -> XY_Translation/2(T2)
  [MOTOR_T3] -> XY_Translation/3(T3)
  [MOTOR_OMEGA_SQ4] -> Yaw_Dynamics/4(omega_sq4)
  XY_Translation/2(y) -> Y_Position_m/1, [TRUE_Y]  "y_true"
  Pitch_Dynamics/1(theta) -> Pitch_rad/1, [TRUE_THETA]  "theta_true"
  Roll_Dynamics/1(phi) -> Roll_rad_Monitor/1, [TRUE_PHI]  "phi_true"
  Motor_3/2(T3) -> V2_Motor_3_Thrust/1, [MOTOR_T3]  "T3"
  Motor_2/2(T2) -> V2_Motor_2_Thrust/1, [MOTOR_T2]  "T2"
  Motor_4/2(T4) -> V2_Motor_4_Thrust/1, [MOTOR_T4]  "T4"
  Motor_Mixer/4(Tcmd4) -> Motor_4/1(Tcmd4), V2_Motor_4_Command/1  "Tcmd4"
  Motor_Mixer/3(Tcmd3) -> Motor_3/1(Tcmd3), V2_Motor_3_Command/1  "Tcmd3"
  Motor_1/2(T1) -> V2_Motor_1_Thrust/1, [MOTOR_T1]  "T1"
  Motor_Mixer/2(Tcmd2) -> Motor_2/1(Tcmd2), V2_Motor_2_Command/1  "Tcmd2"
  Motor_Mixer/1(Tcmd1) -> Motor_1/1(Tcmd1), V2_Motor_1_Command/1  "Tcmd1"
  Motor_1/1(omega_sq1) -> [MOTOR_OMEGA_SQ1]  "omega_sq1"
  Roll_Controller/1(Roll_cmd) -> Motor_Mixer/4(Roll_cmd)  "Roll_cmd"
  Yaw_Controller/1(Yaw_cmd) -> Motor_Mixer/3(Yaw_cmd)  "Yaw_cmd"
  Pitch_Controller/1(Pitch_cmd) -> Motor_Mixer/2(Pitch_cmd)  "Pitch_cmd"
  Select_Collective_Replay/1 -> Motor_Mixer/1(Tbase)  "Tbase_selected"
  Motor_4/1(omega_sq4) -> [MOTOR_OMEGA_SQ4]  "omega_sq4"
  Motor_3/1(omega_sq3) -> [MOTOR_OMEGA_SQ3]  "omega_sq3"
  Motor_2/1(omega_sq2) -> [MOTOR_OMEGA_SQ2]  "omega_sq2"
  Manual_Phase_Enable/1 -> Select_Collective_Replay/2, Select_Roll_Replay/2, Select_Pitch_Replay/2

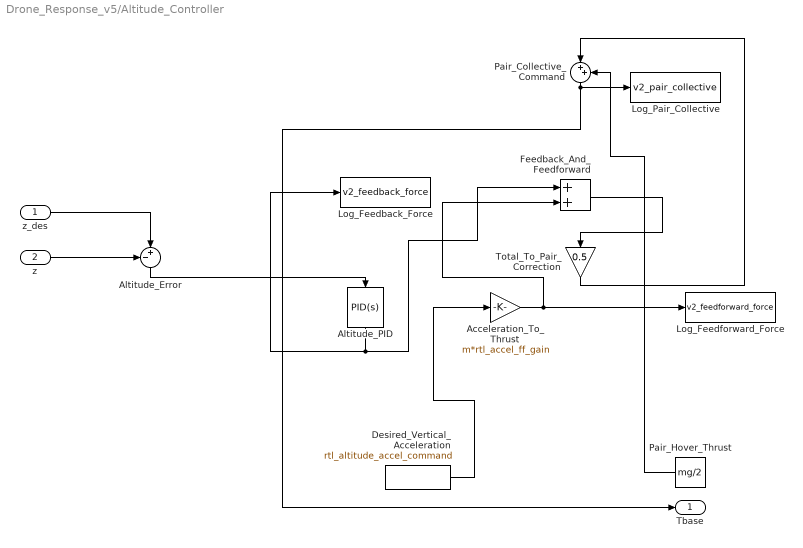
== system Drone_Response_v5/Altitude_Controller ==
  z_des : Inport
  z : Inport  Port=2
  Acceleration_To_Thrust : Gain  Gain=m*rtl_accel_ff_gain
  Altitude_Error : Sum  Inputs=-+|
  Altitude_PID : slpidlib/PID Controller  Controller=PID  Form=Parallel  TimeDomain=Continuous-time  UseExternalTs=off  SampleTime=-1  IntegratorMethod=Forward Euler  FilterMethod=Forward Euler  ControllerParametersSource=internal  P=Kp_z  I=Ki_z  UseKiTs=off  D=Kd_z  UseExternalDerivativeSource=off  N=N_z  UseFilter=on  TunerSelectOption=Transfer Function Based (PID Tuner App)  InitialConditionSource=internal  InitialConditionForIntegrator=0  InitialConditionForFilter=0.00373711537319058  DifferentiatorICPrevScaledInput=0  ExternalReset=none  TrackingMode=off  Kt=1  LimitOutput=off  SatLimitsSource=internal  UpperSaturationLimit=inf  LowerSaturationLimit=-inf  LinearizeAsGain=on  AntiWindupMode=none  Kb=1  LimitIntegrator=off  UpperIntegratorSaturationLimit=inf  LowerIntegratorSaturationLimit=-inf  POutMin=[]  POutMax=[]  IOutMin=[]  IOutMax=[]  DOutMin=[]  DOutMax=[]  NOutMin=[]  NOutMax=[]  SumOutMin=[]  SumOutMax=[]  SaturationOutMin=[]  SaturationOutMax=[]  PParamMin=[]  PParamMax=[]  IParamMin=[]  IParamMax=[]  DParamMin=[]  DParamMax=[]  NParamMin=[]  NParamMax=[]  KbParamMin=[]  KbParamMax=[]  KtParamMin=[]  KtParamMax=[]  KbOutMin=[]  KbOutMax=[]  KtOutMin=[]  KtOutMax=[]  IntegratorOutMin=[]  IntegratorOutMax=[]  FilterOutMin=[]  FilterOutMax=[]  SumI1OutMin=[]  SumI1OutMax=[]  SumI2OutMin=[]  SumI2OutMax=[]  SumI3OutMin=[]  SumI3OutMax=[]  SumI4OutMin=[]  SumI4OutMax=[]  SumDOutMin=[]  SumDOutMax=[]  DifferentiatorOutMin=[]  DifferentiatorOutMax=[]  FilterDiffOutCoefMin=[]  FilterDiffOutCoefMax=[]  ReciprocalOutMin=[]  ReciprocalOutMax=[]  SumDenOutMin=[]  SumDenOutMax=[]  SumNumOutMin=[]  SumNumOutMax=[]  DivideOutMin=[]  DivideOutMax=[]  UdiffTsProdOutMin=[]  UdiffTsProdOutMax=[]  NTsProdOutMin=[]  NTsProdOutMax=[]  UintegralTsProdOutMin=[]  UintegralTsProdOutMax=[]  UngainTsProdOutMin=[]  UngainTsProdOutMax=[]  ClampingZeroOutDataTypeStr=Inherit: Inherit via back propagation  ClampingZeroOutMin=[]  ClampingZeroOutMax=[]  FilterDenConstantOutDataTypeStr=Inherit: Inherit via back propagation  FilterDenConstantOutMin=[]  FilterDenConstantOutMax=[]  PCopyOutDataTypeStr=Inherit: Inherit via back propagation  PCopyOutMin=[]  PCopyOutMax=[]  NCopyOutDataTypeStr=Inherit: Inherit via back propagation  NCopyOutMin=[]  NCopyOutMax=[]  IntegratorContinuousStateAttributes=''  IntegratorStateMustResolveToSignalObject=off  IntegratorRTWStateStorageClass=Auto  FilterContinuousStateAttributes=''  FilterStateMustResolveToSignalObject=off  FilterRTWStateStorageClass=Auto  ParallelPVariant=InternalParameters  IdealPVariant=Disabled  IVariant=InternalParameters  DVariant=InternalParameters  IntegratorVariant=Continuous  SatVariant=Disabled  AWVariant=Passthrough  PCopyVariant=Disabled  TRVariant=Disabled  FdbkBlocksVariant=Forward  IdealPFdbkVariant=Disabled  SatFdbkVariant=Disabled  DerivativeFilterVariant=ContFilter  NVariant=InternalParameters  NCopyVariant=Disabled  FilterICVariant=InternalICsFilter  IntegratorICVariant=InternalICs  ExternalResetVariant=Disabled  TRSumVariant=Passthrough  SumFdbkVariant=Disabled  SumVariant=Sum_PID  TsampFilterVariant=InternalTs  TsampNgainVariant=Passthrough  TsampIntegralVariant=Disabled_SignalSpec  ExternalSaturationOutDataTypeStr=Inherit: Same as second input  DerivativeSourceVariant=ErrorSignal  PreIntVariant=InternalPreInt
  Desired_Vertical_Acceleration : FromWorkspace  VariableName=rtl_altitude_accel_command
  Feedback_And_Feedforward : Sum
  Log_Feedback_Force : ToWorkspace  VariableName=v2_feedback_force  SaveFormat=Timeseries  SampleTime=-1
  Log_Feedforward_Force : ToWorkspace  VariableName=v2_feedforward_force  SaveFormat=Timeseries  SampleTime=-1
  Log_Pair_Collective : ToWorkspace  VariableName=v2_pair_collective  SaveFormat=Timeseries  SampleTime=-1
  Pair_Collective_Command : Sum  Inputs=|++
  Pair_Hover_Thrust : Constant  Value=mg/2
  Total_To_Pair_Correction : Gain  Gain=0.5
  Tbase : Outport
  wires:
  z/1 -> Altitude_Error/1
  z_des/1 -> Altitude_Error/2
  Feedback_And_Feedforward/1 -> Total_To_Pair_Correction/1
  Acceleration_To_Thrust/1 -> Feedback_And_Feedforward/2, Log_Feedforward_Force/1
  Desired_Vertical_Acceleration/1 -> Acceleration_To_Thrust/1
  Altitude_Error/1 -> Altitude_PID/1
  Altitude_PID/1 -> Log_Feedback_Force/1, Feedback_And_Feedforward/1
  Total_To_Pair_Correction/1 -> Pair_Collective_Command/1
  Pair_Collective_Command/1 -> Log_Pair_Collective/1, Tbase/1
  Pair_Hover_Thrust/1 -> Pair_Collective_Command/2

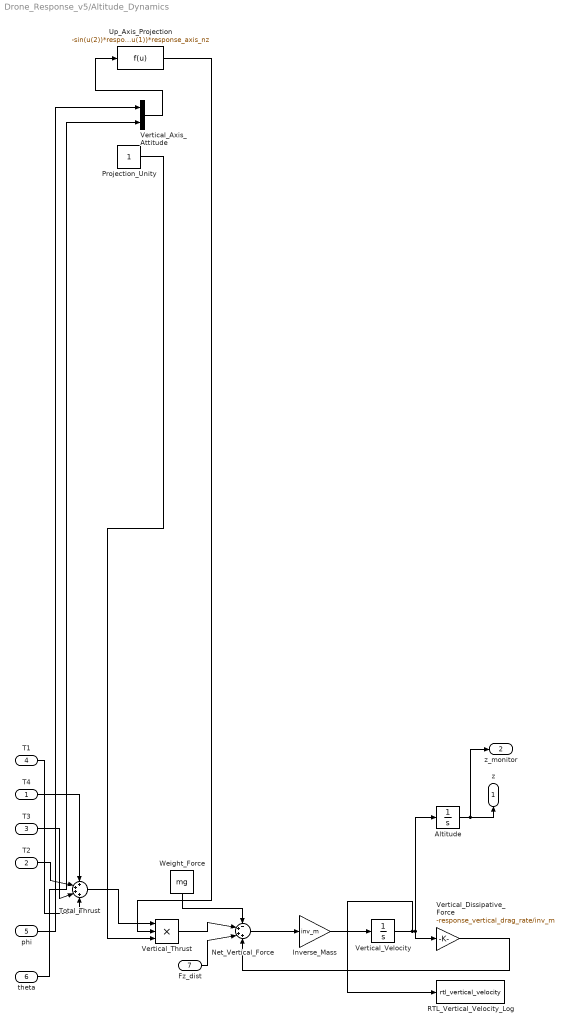
== system Drone_Response_v5/Altitude_Dynamics ==
  T4 : Inport
  T2 : Inport  Port=2
  T3 : Inport  Port=3
  T1 : Inport  Port=4
  phi : Inport  Port=5
  theta : Inport  Port=6
  Fz_dist : Inport  Port=7
  Altitude : Integrator  InitialCondition=z0
  Inverse_Mass : Gain  Gain=inv_m
  Net_Vertical_Force : Sum  Inputs=-+++
  Projection_Unity : Constant
  RTL_Vertical_Velocity_Log : ToWorkspace  VariableName=rtl_vertical_velocity  SaveFormat=Timeseries  SampleTime=-1
  Total_Thrust : Sum  Inputs=++++
  Up_Axis_Projection : Fcn  Expr=-sin(u(2))*response_axis_nx+cos(u(2))*sin(u(1))*response_axis_ny+cos(u(2))*cos(u(1))*response_axis_nz
  Vertical_Axis_Attitude : Mux  Inputs=2
  Vertical_Dissipative_Force : Gain  Gain=-response_vertical_drag_rate/inv_m
  Vertical_Thrust : Product  Inputs=3
  Vertical_Velocity : Integrator  InitialCondition=vz0
  Weight_Force : Constant  Value=mg
  z : Outport
  z_monitor : Outport  Port=2
  wires:
  T1/1 -> Total_Thrust/4
  T2/1 -> Total_Thrust/2
  Weight_Force/1 -> Net_Vertical_Force/1
  T4/1 -> Total_Thrust/1
  T3/1 -> Total_Thrust/3
  Total_Thrust/1 -> Vertical_Thrust/1
  Vertical_Thrust/1 -> Net_Vertical_Force/2
  Net_Vertical_Force/1 -> Inverse_Mass/1
  Inverse_Mass/1 -> Vertical_Velocity/1
  Fz_dist/1 -> Net_Vertical_Force/3
  Vertical_Dissipative_Force/1 -> Net_Vertical_Force/4
  Vertical_Velocity/1 -> Vertical_Dissipative_Force/1, Altitude/1, RTL_Vertical_Velocity_Log/1
  Altitude/1 -> z/1, z_monitor/1
  phi/1 -> Vertical_Axis_Attitude/1
  theta/1 -> Vertical_Axis_Attitude/2
  Vertical_Axis_Attitude/1 -> Up_Axis_Projection/1
  Up_Axis_Projection/1 -> Vertical_Thrust/2
  Projection_Unity/1 -> Vertical_Thrust/3

== system Drone_Response_v5/Attitude_Mode_Selector ==
  mode : Inport
  phi_manual : Inport  Port=2
  theta_manual : Inport  Port=3
  phi_position : Inport  Port=4
  theta_position : Inport  Port=5
  Select_Pitch_Command : Switch  Threshold=1.5  SaturateOnIntegerOverflow=off  InputSameDT=off
  Select_Roll_Command : Switch  Threshold=1.5  SaturateOnIntegerOverflow=off  InputSameDT=off
  phi_des : Outport
  theta_des : Outport  Port=2
  wires:
  [ATTITUDE_MODE] -> Select_Pitch_Command/2
  [ATTITUDE_MODE] -> Select_Roll_Command/2
  phi_position/1 -> Select_Roll_Command/1
  mode/1 -> [ATTITUDE_MODE]
  phi_manual/1 -> Select_Roll_Command/3
  Select_Roll_Command/1 -> phi_des/1
  theta_position/1 -> Select_Pitch_Command/1
  theta_manual/1 -> Select_Pitch_Command/3
  Select_Pitch_Command/1 -> theta_des/1

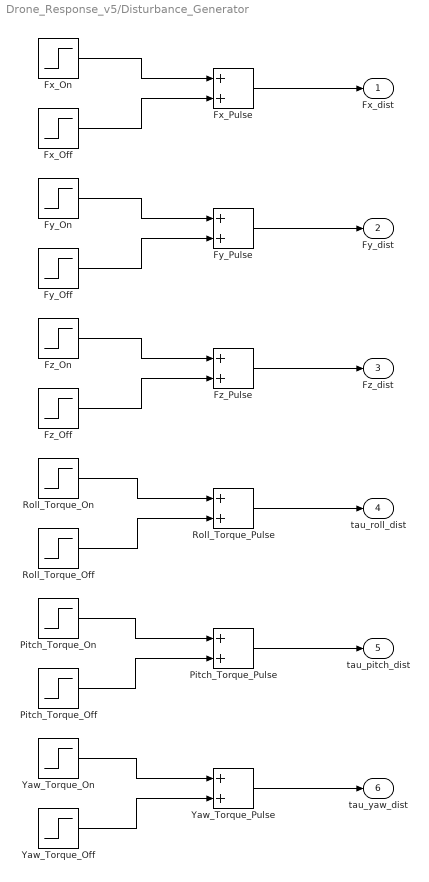
== system Drone_Response_v5/Disturbance_Generator ==
  Fx_Off : Step  Time=t_Fx_end  After=-disturbances_enabled*Fx_gust  SampleTime=0
  Fx_On : Step  Time=t_Fx_start  After=disturbances_enabled*Fx_gust  SampleTime=0
  Fx_Pulse : Sum
  Fy_Off : Step  Time=t_Fy_end  After=-disturbances_enabled*Fy_gust  SampleTime=0
  Fy_On : Step  Time=t_Fy_start  After=disturbances_enabled*Fy_gust  SampleTime=0
  Fy_Pulse : Sum
  Fz_Off : Step  Time=t_Fz_end  After=-disturbances_enabled*Fz_gust  SampleTime=0
  Fz_On : Step  Time=t_Fz_start  After=disturbances_enabled*Fz_gust  SampleTime=0
  Fz_Pulse : Sum
  Pitch_Torque_Off : Step  Time=t_pitch_end  After=-disturbances_enabled*tau_pitch_gust  SampleTime=0
  Pitch_Torque_On : Step  Time=t_pitch_start  After=disturbances_enabled*tau_pitch_gust  SampleTime=0
  Pitch_Torque_Pulse : Sum
  Roll_Torque_Off : Step  Time=t_roll_end  After=-disturbances_enabled*tau_roll_gust  SampleTime=0
  Roll_Torque_On : Step  Time=t_roll_start  After=disturbances_enabled*tau_roll_gust  SampleTime=0
  Roll_Torque_Pulse : Sum
  Yaw_Torque_Off : Step  Time=t_yaw_end  After=-disturbances_enabled*tau_yaw_gust  SampleTime=0
  Yaw_Torque_On : Step  Time=t_yaw_start  After=disturbances_enabled*tau_yaw_gust  SampleTime=0
  Yaw_Torque_Pulse : Sum
  Fx_dist : Outport
  Fy_dist : Outport  Port=2
  Fz_dist : Outport  Port=3
  tau_roll_dist : Outport  Port=4
  tau_pitch_dist : Outport  Port=5
  tau_yaw_dist : Outport  Port=6
  wires:
  Yaw_Torque_Pulse/1 -> tau_yaw_dist/1
  Yaw_Torque_Off/1 -> Yaw_Torque_Pulse/2
  Yaw_Torque_On/1 -> Yaw_Torque_Pulse/1
  Pitch_Torque_Pulse/1 -> tau_pitch_dist/1
  Pitch_Torque_Off/1 -> Pitch_Torque_Pulse/2
  Pitch_Torque_On/1 -> Pitch_Torque_Pulse/1
  Roll_Torque_Pulse/1 -> tau_roll_dist/1
  Roll_Torque_Off/1 -> Roll_Torque_Pulse/2
  Roll_Torque_On/1 -> Roll_Torque_Pulse/1
  Fz_Pulse/1 -> Fz_dist/1
  Fz_Off/1 -> Fz_Pulse/2
  Fz_On/1 -> Fz_Pulse/1
  Fy_Pulse/1 -> Fy_dist/1
  Fy_Off/1 -> Fy_Pulse/2
  Fy_On/1 -> Fy_Pulse/1
  Fx_Pulse/1 -> Fx_dist/1
  Fx_Off/1 -> Fx_Pulse/2
  Fx_On/1 -> Fx_Pulse/1

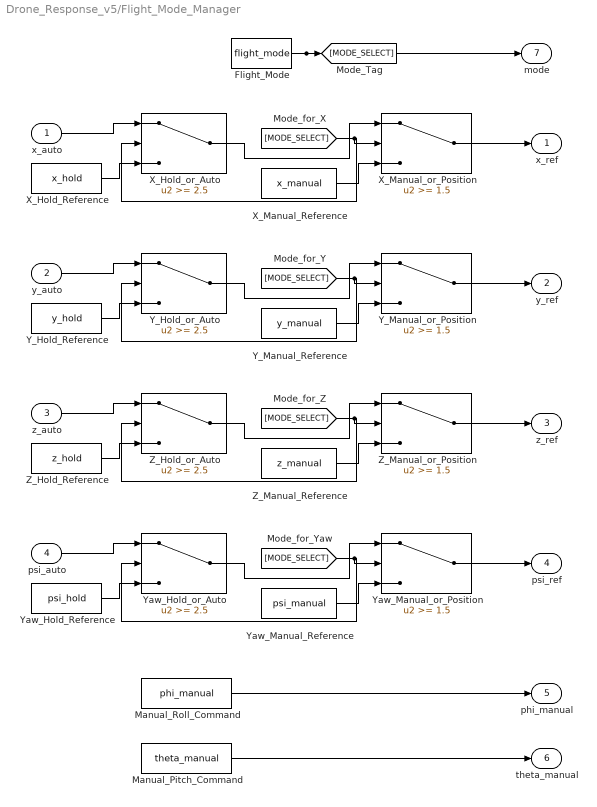
== system Drone_Response_v5/Flight_Mode_Manager ==
  x_auto : Inport
  y_auto : Inport  Port=2
  z_auto : Inport  Port=3
  psi_auto : Inport  Port=4
  Flight_Mode : Constant  Value=flight_mode
  Manual_Pitch_Command : Constant  Value=theta_manual
  Manual_Roll_Command : Constant  Value=phi_manual
  X_Hold_Reference : Constant  Value=x_hold
  X_Hold_or_Auto : Switch  Threshold=2.5  SaturateOnIntegerOverflow=off  InputSameDT=off
  X_Manual_Reference : Constant  Value=x_manual
  X_Manual_or_Position : Switch  Threshold=1.5  SaturateOnIntegerOverflow=off  InputSameDT=off
  Y_Hold_Reference : Constant  Value=y_hold
  Y_Hold_or_Auto : Switch  Threshold=2.5  SaturateOnIntegerOverflow=off  InputSameDT=off
  Y_Manual_Reference : Constant  Value=y_manual
  Y_Manual_or_Position : Switch  Threshold=1.5  SaturateOnIntegerOverflow=off  InputSameDT=off
  Yaw_Hold_Reference : Constant  Value=psi_hold
  Yaw_Hold_or_Auto : Switch  Threshold=2.5  SaturateOnIntegerOverflow=off  InputSameDT=off
  Yaw_Manual_Reference : Constant  Value=psi_manual
  Yaw_Manual_or_Position : Switch  Threshold=1.5  SaturateOnIntegerOverflow=off  InputSameDT=off
  Z_Hold_Reference : Constant  Value=z_hold
  Z_Hold_or_Auto : Switch  Threshold=2.5  SaturateOnIntegerOverflow=off  InputSameDT=off
  Z_Manual_Reference : Constant  Value=z_manual
  Z_Manual_or_Position : Switch  Threshold=1.5  SaturateOnIntegerOverflow=off  InputSameDT=off
  x_ref : Outport
  y_ref : Outport  Port=2
  z_ref : Outport  Port=3
  psi_ref : Outport  Port=4
  phi_manual : Outport  Port=5
  theta_manual : Outport  Port=6
  mode : Outport  Port=7
  wires:
  [MODE_SELECT] -> Yaw_Hold_or_Auto/2, Yaw_Manual_or_Position/2
  [MODE_SELECT] -> Z_Hold_or_Auto/2, Z_Manual_or_Position/2
  [MODE_SELECT] -> Y_Hold_or_Auto/2, Y_Manual_or_Position/2
  [MODE_SELECT] -> X_Hold_or_Auto/2, X_Manual_or_Position/2
  x_auto/1 -> X_Hold_or_Auto/1
  Flight_Mode/1 -> mode/1, [MODE_SELECT]
  X_Hold_Reference/1 -> X_Hold_or_Auto/3
  X_Hold_or_Auto/1 -> X_Manual_or_Position/1
  X_Manual_Reference/1 -> X_Manual_or_Position/3
  X_Manual_or_Position/1 -> x_ref/1
  y_auto/1 -> Y_Hold_or_Auto/1
  Y_Hold_Reference/1 -> Y_Hold_or_Auto/3
  Y_Hold_or_Auto/1 -> Y_Manual_or_Position/1
  Y_Manual_Reference/1 -> Y_Manual_or_Position/3
  Y_Manual_or_Position/1 -> y_ref/1
  z_auto/1 -> Z_Hold_or_Auto/1
  Z_Hold_Reference/1 -> Z_Hold_or_Auto/3
  Z_Hold_or_Auto/1 -> Z_Manual_or_Position/1
  Z_Manual_Reference/1 -> Z_Manual_or_Position/3
  Z_Manual_or_Position/1 -> z_ref/1
  psi_auto/1 -> Yaw_Hold_or_Auto/1
  Yaw_Hold_Reference/1 -> Yaw_Hold_or_Auto/3
  Yaw_Hold_or_Auto/1 -> Yaw_Manual_or_Position/1
  Yaw_Manual_Reference/1 -> Yaw_Manual_or_Position/3
  Yaw_Manual_or_Position/1 -> psi_ref/1
  Manual_Roll_Command/1 -> phi_manual/1
  Manual_Pitch_Command/1 -> theta_manual/1

== system Drone_Response_v5/Motor_1 ==
  Tcmd1 : Inport
  Commanded_Rotor_Speed : Sqrt
  Inverse_Motor_Time_Constant : Gain  Gain=1/tau_m
  Inverse_Thrust_Coefficient : Gain  Gain=1/kf
  Rotor_Speed : Integrator  InitialCondition=omega_init
  Rotor_Speed_Error : Sum  Inputs=|+-
  Rotor_Speed_Squared : Math  Operator=square
  Thrust_Coefficient : Gain  Gain=kf
  Thrust_Limit : Saturate  UpperLimit=Tmax  LowerLimit=Tmin
  omega_sq1 : Outport
  T1 : Outport  Port=2
  wires:
  Tcmd1/1 -> Thrust_Limit/1
  Rotor_Speed/1 -> Rotor_Speed_Error/2, Rotor_Speed_Squared/1
  Inverse_Motor_Time_Constant/1 -> Rotor_Speed/1
  Inverse_Thrust_Coefficient/1 -> Commanded_Rotor_Speed/1
  Rotor_Speed_Error/1 -> Inverse_Motor_Time_Constant/1
  Rotor_Speed_Squared/1 -> Thrust_Coefficient/1, omega_sq1/1
  Commanded_Rotor_Speed/1 -> Rotor_Speed_Error/1
  Thrust_Limit/1 -> Inverse_Thrust_Coefficient/1
  Thrust_Coefficient/1 -> T1/1

== system Drone_Response_v5/Motor_2 ==
  Tcmd2 : Inport
  Commanded_Rotor_Speed : Sqrt
  Inverse_Motor_Time_Constant : Gain  Gain=1/tau_m
  Inverse_Thrust_Coefficient : Gain  Gain=1/kf
  Rotor_Speed : Integrator  InitialCondition=omega_init
  Rotor_Speed_Error : Sum  Inputs=|+-
  Rotor_Speed_Squared : Math  Operator=square
  Thrust_Coefficient : Gain  Gain=kf
  Thrust_Limit : Saturate  UpperLimit=Tmax  LowerLimit=Tmin
  omega_sq2 : Outport
  T2 : Outport  Port=2
  wires:
  Tcmd2/1 -> Thrust_Limit/1
  Rotor_Speed/1 -> Rotor_Speed_Error/2, Rotor_Speed_Squared/1
  Inverse_Motor_Time_Constant/1 -> Rotor_Speed/1
  Inverse_Thrust_Coefficient/1 -> Commanded_Rotor_Speed/1
  Rotor_Speed_Squared/1 -> omega_sq2/1, Thrust_Coefficient/1
  Commanded_Rotor_Speed/1 -> Rotor_Speed_Error/1
  Rotor_Speed_Error/1 -> Inverse_Motor_Time_Constant/1
  Thrust_Limit/1 -> Inverse_Thrust_Coefficient/1
  Thrust_Coefficient/1 -> T2/1

== system Drone_Response_v5/Motor_3 ==
  Tcmd3 : Inport
  Commanded_Rotor_Speed : Sqrt
  Inverse_Motor_Time_Constant : Gain  Gain=1/tau_m
  Inverse_Thrust_Coefficient : Gain  Gain=1/kf
  Rotor_Speed : Integrator  InitialCondition=omega_init
  Rotor_Speed_Error : Sum  Inputs=|+-
  Rotor_Speed_Squared : Math  Operator=square
  Thrust_Coefficient : Gain  Gain=kf
  Thrust_Limit : Saturate  UpperLimit=Tmax  LowerLimit=Tmin
  omega_sq3 : Outport
  T3 : Outport  Port=2
  wires:
  Rotor_Speed_Squared/1 -> omega_sq3/1, Thrust_Coefficient/1
  Rotor_Speed/1 -> Rotor_Speed_Error/2, Rotor_Speed_Squared/1
  Inverse_Motor_Time_Constant/1 -> Rotor_Speed/1
  Thrust_Coefficient/1 -> T3/1
  Rotor_Speed_Error/1 -> Inverse_Motor_Time_Constant/1
  Commanded_Rotor_Speed/1 -> Rotor_Speed_Error/1
  Inverse_Thrust_Coefficient/1 -> Commanded_Rotor_Speed/1
  Thrust_Limit/1 -> Inverse_Thrust_Coefficient/1
  Tcmd3/1 -> Thrust_Limit/1

== system Drone_Response_v5/Motor_4 ==
  Tcmd4 : Inport
  Commanded_Rotor_Speed : Sqrt
  Inverse_Motor_Time_Constant : Gain  Gain=1/tau_m
  Inverse_Thrust_Coefficient : Gain  Gain=1/kf
  Rotor_Speed : Integrator  InitialCondition=omega_init
  Rotor_Speed_Error : Sum  Inputs=|+-
  Rotor_Speed_Squared : Math  Operator=square
  Thrust_Coefficient : Gain  Gain=kf
  Thrust_Limit : Saturate  UpperLimit=Tmax  LowerLimit=Tmin
  omega_sq4 : Outport
  T4 : Outport  Port=2
  wires:
  Rotor_Speed/1 -> Rotor_Speed_Error/2, Rotor_Speed_Squared/1
  Inverse_Motor_Time_Constant/1 -> Rotor_Speed/1
  Inverse_Thrust_Coefficient/1 -> Commanded_Rotor_Speed/1
  Tcmd4/1 -> Thrust_Limit/1
  Rotor_Speed_Squared/1 -> omega_sq4/1, Thrust_Coefficient/1
  Rotor_Speed_Error/1 -> Inverse_Motor_Time_Constant/1
  Commanded_Rotor_Speed/1 -> Rotor_Speed_Error/1
  Thrust_Limit/1 -> Inverse_Thrust_Coefficient/1
  Thrust_Coefficient/1 -> T4/1

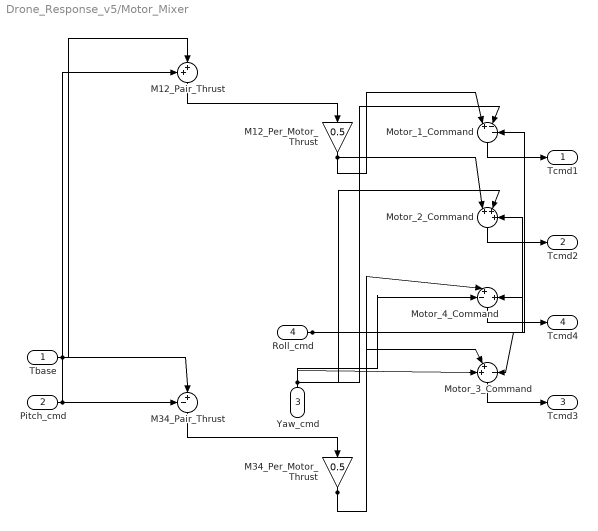
== system Drone_Response_v5/Motor_Mixer ==
  Tbase : Inport
  Pitch_cmd : Inport  Port=2
  Yaw_cmd : Inport  Port=3
  Roll_cmd : Inport  Port=4
  M12_Pair_Thrust : Sum  Inputs=++|
  M12_Per_Motor_Thrust : Gain  Gain=0.5
  M34_Pair_Thrust : Sum  Inputs=-+|
  M34_Per_Motor_Thrust : Gain  Gain=0.5
  Motor_1_Command : Sum  Inputs=|+--
  Motor_2_Command : Sum  Inputs=|+++
  Motor_3_Command : Sum  Inputs=++|-
  Motor_4_Command : Sum  Inputs=-+|+
  Tcmd1 : Outport
  Tcmd2 : Outport  Port=2
  Tcmd3 : Outport  Port=3
  Tcmd4 : Outport  Port=4
  wires:
  M34_Per_Motor_Thrust/1 -> Motor_4_Command/2, Motor_3_Command/2
  Yaw_cmd/1 -> Motor_1_Command/2, Motor_2_Command/2, Motor_3_Command/1, Motor_4_Command/1
  Roll_cmd/1 -> Motor_4_Command/3, Motor_3_Command/3, Motor_2_Command/3, Motor_1_Command/3
  M12_Per_Motor_Thrust/1 -> Motor_2_Command/1, Motor_1_Command/1
  Pitch_cmd/1 -> M12_Pair_Thrust/1, M34_Pair_Thrust/1
  Motor_1_Command/1 -> Tcmd1/1
  Tbase/1 -> M34_Pair_Thrust/2, M12_Pair_Thrust/2
  M34_Pair_Thrust/1 -> M34_Per_Motor_Thrust/1
  M12_Pair_Thrust/1 -> M12_Per_Motor_Thrust/1
  Motor_2_Command/1 -> Tcmd2/1
  Motor_4_Command/1 -> Tcmd4/1
  Motor_3_Command/1 -> Tcmd3/1

== system Drone_Response_v5/Pitch_Controller ==
  theta_des : Inport
  theta : Inport  Port=2
  Pitch_Error : Sum  Inputs=|+-
  Pitch_PID : slpidlib/PID Controller  Controller=PID  Form=Parallel  TimeDomain=Continuous-time  UseExternalTs=off  SampleTime=-1  IntegratorMethod=Forward Euler  FilterMethod=Forward Euler  ControllerParametersSource=internal  P=Kp_theta  I=Ki_theta  UseKiTs=off  D=Kd_theta  UseExternalDerivativeSource=off  N=N_theta  UseFilter=on  TunerSelectOption=Transfer Function Based (PID Tuner App)  InitialConditionSource=internal  InitialConditionForIntegrator=0  InitialConditionForFilter=-0.00816417634149544  DifferentiatorICPrevScaledInput=0  ExternalReset=none  TrackingMode=off  Kt=1  LimitOutput=off  SatLimitsSource=internal  UpperSaturationLimit=inf  LowerSaturationLimit=-inf  LinearizeAsGain=on  AntiWindupMode=none  Kb=1  LimitIntegrator=off  UpperIntegratorSaturationLimit=inf  LowerIntegratorSaturationLimit=-inf  POutMin=[]  POutMax=[]  IOutMin=[]  IOutMax=[]  DOutMin=[]  DOutMax=[]  NOutMin=[]  NOutMax=[]  SumOutMin=[]  SumOutMax=[]  SaturationOutMin=[]  SaturationOutMax=[]  PParamMin=[]  PParamMax=[]  IParamMin=[]  IParamMax=[]  DParamMin=[]  DParamMax=[]  NParamMin=[]  NParamMax=[]  KbParamMin=[]  KbParamMax=[]  KtParamMin=[]  KtParamMax=[]  KbOutMin=[]  KbOutMax=[]  KtOutMin=[]  KtOutMax=[]  IntegratorOutMin=[]  IntegratorOutMax=[]  FilterOutMin=[]  FilterOutMax=[]  SumI1OutMin=[]  SumI1OutMax=[]  SumI2OutMin=[]  SumI2OutMax=[]  SumI3OutMin=[]  SumI3OutMax=[]  SumI4OutMin=[]  SumI4OutMax=[]  SumDOutMin=[]  SumDOutMax=[]  DifferentiatorOutMin=[]  DifferentiatorOutMax=[]  FilterDiffOutCoefMin=[]  FilterDiffOutCoefMax=[]  ReciprocalOutMin=[]  ReciprocalOutMax=[]  SumDenOutMin=[]  SumDenOutMax=[]  SumNumOutMin=[]  SumNumOutMax=[]  DivideOutMin=[]  DivideOutMax=[]  UdiffTsProdOutMin=[]  UdiffTsProdOutMax=[]  NTsProdOutMin=[]  NTsProdOutMax=[]  UintegralTsProdOutMin=[]  UintegralTsProdOutMax=[]  UngainTsProdOutMin=[]  UngainTsProdOutMax=[]  ClampingZeroOutDataTypeStr=Inherit: Inherit via back propagation  ClampingZeroOutMin=[]  ClampingZeroOutMax=[]  FilterDenConstantOutDataTypeStr=Inherit: Inherit via back propagation  FilterDenConstantOutMin=[]  FilterDenConstantOutMax=[]  PCopyOutDataTypeStr=Inherit: Inherit via back propagation  PCopyOutMin=[]  PCopyOutMax=[]  NCopyOutDataTypeStr=Inherit: Inherit via back propagation  NCopyOutMin=[]  NCopyOutMax=[]  IntegratorContinuousStateAttributes=''  IntegratorStateMustResolveToSignalObject=off  IntegratorRTWStateStorageClass=Auto  FilterContinuousStateAttributes=''  FilterStateMustResolveToSignalObject=off  FilterRTWStateStorageClass=Auto  ParallelPVariant=InternalParameters  IdealPVariant=Disabled  IVariant=InternalParameters  DVariant=InternalParameters  IntegratorVariant=Continuous  SatVariant=Disabled  AWVariant=Passthrough  PCopyVariant=Disabled  TRVariant=Disabled  FdbkBlocksVariant=Forward  IdealPFdbkVariant=Disabled  SatFdbkVariant=Disabled  DerivativeFilterVariant=ContFilter  NVariant=InternalParameters  NCopyVariant=Disabled  FilterICVariant=InternalICsFilter  IntegratorICVariant=InternalICs  ExternalResetVariant=Disabled  TRSumVariant=Passthrough  SumFdbkVariant=Disabled  SumVariant=Sum_PID  TsampFilterVariant=InternalTs  TsampNgainVariant=Passthrough  TsampIntegralVariant=Disabled_SignalSpec  ExternalSaturationOutDataTypeStr=Inherit: Same as second input  DerivativeSourceVariant=ErrorSignal  PreIntVariant=InternalPreInt
  Pitch_Pair_Allocation : Gain  Gain=pitch_pair_allocation
  Pitch_cmd : Outport
  wires:
  Pitch_Pair_Allocation/1 -> Pitch_cmd/1
  Pitch_PID/1 -> Pitch_Pair_Allocation/1
  Pitch_Error/1 -> Pitch_PID/1
  theta/1 -> Pitch_Error/2
  theta_des/1 -> Pitch_Error/1

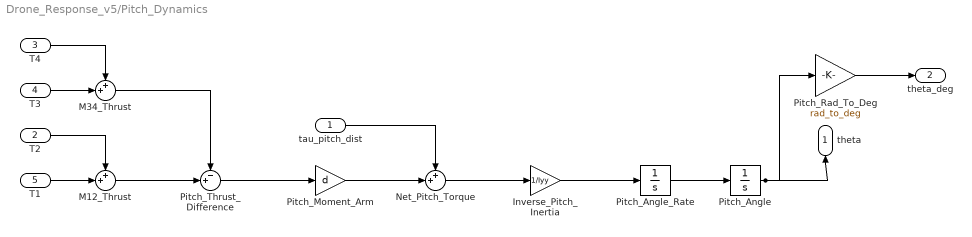
== system Drone_Response_v5/Pitch_Dynamics ==
  tau_pitch_dist : Inport
  T2 : Inport  Port=2
  T4 : Inport  Port=3
  T3 : Inport  Port=4
  T1 : Inport  Port=5
  Inverse_Pitch_Inertia : Gain  Gain=1/Iyy
  M12_Thrust : Sum  Inputs=++|
  M34_Thrust : Sum  Inputs=++|
  Net_Pitch_Torque : Sum  Inputs=++|
  Pitch_Angle : Integrator  InitialCondition=theta0
  Pitch_Angle_Rate : Integrator  InitialCondition=theta_dot0
  Pitch_Moment_Arm : Gain  Gain=d
  Pitch_Rad_To_Deg : Gain  Gain=rad_to_deg
  Pitch_Thrust_Difference : Sum  Inputs=-+|
  theta : Outport
  theta_deg : Outport  Port=2
  wires:
  Pitch_Angle/1 -> Pitch_Rad_To_Deg/1, theta/1
  Pitch_Thrust_Difference/1 -> Pitch_Moment_Arm/1
  T1/1 -> M12_Thrust/2
  T2/1 -> M12_Thrust/1
  Pitch_Rad_To_Deg/1 -> theta_deg/1
  T3/1 -> M34_Thrust/2
  Pitch_Angle_Rate/1 -> Pitch_Angle/1
  T4/1 -> M34_Thrust/1
  M12_Thrust/1 -> Pitch_Thrust_Difference/2
  M34_Thrust/1 -> Pitch_Thrust_Difference/1
  tau_pitch_dist/1 -> Net_Pitch_Torque/1
  Pitch_Moment_Arm/1 -> Net_Pitch_Torque/2
  Inverse_Pitch_Inertia/1 -> Pitch_Angle_Rate/1
  Net_Pitch_Torque/1 -> Inverse_Pitch_Inertia/1

== system Drone_Response_v5/Roll_Controller ==
  phi_des : Inport
  phi : Inport  Port=2
  Roll_Error : Sum  Inputs=|+-
  Roll_Motor_Allocation : Gain  Gain=roll_motor_allocation
  Roll_PID : slpidlib/PID Controller  Controller=PID  Form=Parallel  TimeDomain=Continuous-time  UseExternalTs=off  SampleTime=-1  IntegratorMethod=Forward Euler  FilterMethod=Forward Euler  ControllerParametersSource=internal  P=Kp_phi  I=Ki_phi  UseKiTs=off  D=Kd_phi  UseExternalDerivativeSource=off  N=N_phi  UseFilter=on  TunerSelectOption=Transfer Function Based (PID Tuner App)  InitialConditionSource=internal  InitialConditionForIntegrator=0  InitialConditionForFilter=-0.00546025164574833  DifferentiatorICPrevScaledInput=0  ExternalReset=none  TrackingMode=off  Kt=1  LimitOutput=off  SatLimitsSource=internal  UpperSaturationLimit=inf  LowerSaturationLimit=-inf  LinearizeAsGain=on  AntiWindupMode=none  Kb=1  LimitIntegrator=off  UpperIntegratorSaturationLimit=inf  LowerIntegratorSaturationLimit=-inf  POutMin=[]  POutMax=[]  IOutMin=[]  IOutMax=[]  DOutMin=[]  DOutMax=[]  NOutMin=[]  NOutMax=[]  SumOutMin=[]  SumOutMax=[]  SaturationOutMin=[]  SaturationOutMax=[]  PParamMin=[]  PParamMax=[]  IParamMin=[]  IParamMax=[]  DParamMin=[]  DParamMax=[]  NParamMin=[]  NParamMax=[]  KbParamMin=[]  KbParamMax=[]  KtParamMin=[]  KtParamMax=[]  KbOutMin=[]  KbOutMax=[]  KtOutMin=[]  KtOutMax=[]  IntegratorOutMin=[]  IntegratorOutMax=[]  FilterOutMin=[]  FilterOutMax=[]  SumI1OutMin=[]  SumI1OutMax=[]  SumI2OutMin=[]  SumI2OutMax=[]  SumI3OutMin=[]  SumI3OutMax=[]  SumI4OutMin=[]  SumI4OutMax=[]  SumDOutMin=[]  SumDOutMax=[]  DifferentiatorOutMin=[]  DifferentiatorOutMax=[]  FilterDiffOutCoefMin=[]  FilterDiffOutCoefMax=[]  ReciprocalOutMin=[]  ReciprocalOutMax=[]  SumDenOutMin=[]  SumDenOutMax=[]  SumNumOutMin=[]  SumNumOutMax=[]  DivideOutMin=[]  DivideOutMax=[]  UdiffTsProdOutMin=[]  UdiffTsProdOutMax=[]  NTsProdOutMin=[]  NTsProdOutMax=[]  UintegralTsProdOutMin=[]  UintegralTsProdOutMax=[]  UngainTsProdOutMin=[]  UngainTsProdOutMax=[]  ClampingZeroOutDataTypeStr=Inherit: Inherit via back propagation  ClampingZeroOutMin=[]  ClampingZeroOutMax=[]  FilterDenConstantOutDataTypeStr=Inherit: Inherit via back propagation  FilterDenConstantOutMin=[]  FilterDenConstantOutMax=[]  PCopyOutDataTypeStr=Inherit: Inherit via back propagation  PCopyOutMin=[]  PCopyOutMax=[]  NCopyOutDataTypeStr=Inherit: Inherit via back propagation  NCopyOutMin=[]  NCopyOutMax=[]  IntegratorContinuousStateAttributes=''  IntegratorStateMustResolveToSignalObject=off  IntegratorRTWStateStorageClass=Auto  FilterContinuousStateAttributes=''  FilterStateMustResolveToSignalObject=off  FilterRTWStateStorageClass=Auto  ParallelPVariant=InternalParameters  IdealPVariant=Disabled  IVariant=InternalParameters  DVariant=InternalParameters  IntegratorVariant=Continuous  SatVariant=Disabled  AWVariant=Passthrough  PCopyVariant=Disabled  TRVariant=Disabled  FdbkBlocksVariant=Forward  IdealPFdbkVariant=Disabled  SatFdbkVariant=Disabled  DerivativeFilterVariant=ContFilter  NVariant=InternalParameters  NCopyVariant=Disabled  FilterICVariant=InternalICsFilter  IntegratorICVariant=InternalICs  ExternalResetVariant=Disabled  TRSumVariant=Passthrough  SumFdbkVariant=Disabled  SumVariant=Sum_PID  TsampFilterVariant=InternalTs  TsampNgainVariant=Passthrough  TsampIntegralVariant=Disabled_SignalSpec  ExternalSaturationOutDataTypeStr=Inherit: Same as second input  DerivativeSourceVariant=ErrorSignal  PreIntVariant=InternalPreInt
  Roll_cmd : Outport
  wires:
  Roll_Motor_Allocation/1 -> Roll_cmd/1
  Roll_PID/1 -> Roll_Motor_Allocation/1
  Roll_Error/1 -> Roll_PID/1
  phi/1 -> Roll_Error/2
  phi_des/1 -> Roll_Error/1

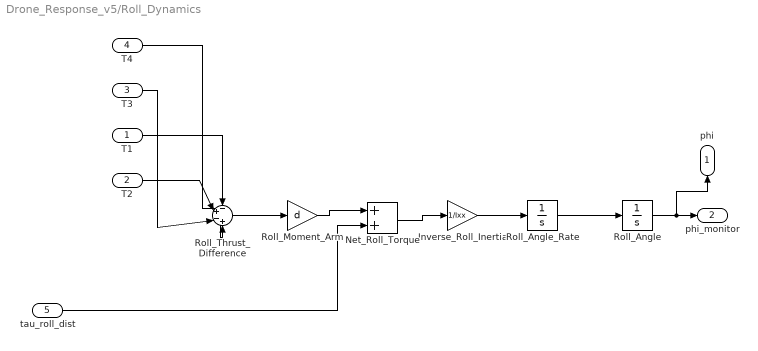
== system Drone_Response_v5/Roll_Dynamics ==
  T1 : Inport
  T2 : Inport  Port=2
  T3 : Inport  Port=3
  T4 : Inport  Port=4
  tau_roll_dist : Inport  Port=5
  Inverse_Roll_Inertia : Gain  Gain=1/Ixx
  Net_Roll_Torque : Sum
  Roll_Angle : Integrator  InitialCondition=phi0
  Roll_Angle_Rate : Integrator  InitialCondition=phi_dot0
  Roll_Moment_Arm : Gain  Gain=d
  Roll_Thrust_Difference : Sum  Inputs=-+-+
  phi : Outport
  phi_monitor : Outport  Port=2
  wires:
  T2/1 -> Roll_Thrust_Difference/2
  T1/1 -> Roll_Thrust_Difference/1
  T3/1 -> Roll_Thrust_Difference/3
  T4/1 -> Roll_Thrust_Difference/4
  Inverse_Roll_Inertia/1 -> Roll_Angle_Rate/1
  Net_Roll_Torque/1 -> Inverse_Roll_Inertia/1
  tau_roll_dist/1 -> Net_Roll_Torque/2
  Roll_Moment_Arm/1 -> Net_Roll_Torque/1
  Roll_Thrust_Difference/1 -> Roll_Moment_Arm/1
  Roll_Angle_Rate/1 -> Roll_Angle/1
  Roll_Angle/1 -> phi/1, phi_monitor/1

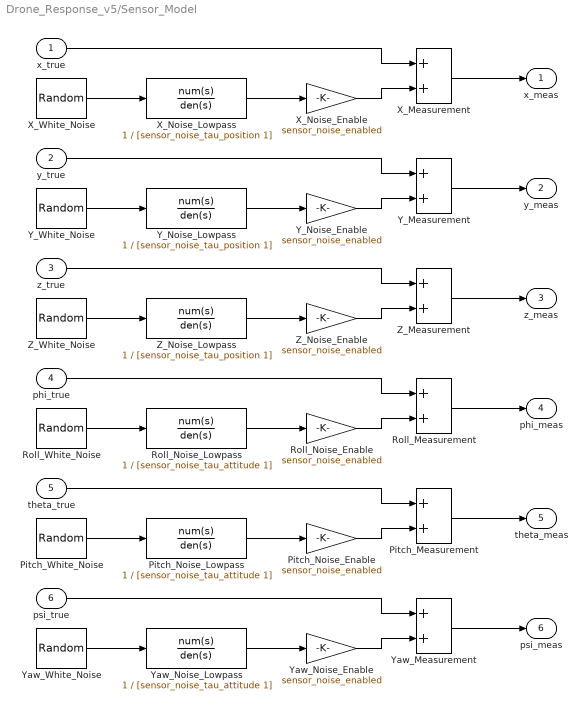
== system Drone_Response_v5/Sensor_Model ==
  x_true : Inport
  y_true : Inport  Port=2
  z_true : Inport  Port=3
  phi_true : Inport  Port=4
  theta_true : Inport  Port=5
  psi_true : Inport  Port=6
  Pitch_Measurement : Sum
  Pitch_Noise_Enable : Gain  Gain=sensor_noise_enabled
  Pitch_Noise_Lowpass : TransferFcn  Numerator=1  Denominator=[sensor_noise_tau_attitude 1]
  Pitch_White_Noise : RandomNumber  Variance=sigma_theta^2  Seed=seed_theta  SampleTime=sensor_sample_time
  Roll_Measurement : Sum
  Roll_Noise_Enable : Gain  Gain=sensor_noise_enabled
  Roll_Noise_Lowpass : TransferFcn  Numerator=1  Denominator=[sensor_noise_tau_attitude 1]
  Roll_White_Noise : RandomNumber  Variance=sigma_phi^2  Seed=seed_phi  SampleTime=sensor_sample_time
  X_Measurement : Sum
  X_Noise_Enable : Gain  Gain=sensor_noise_enabled
  X_Noise_Lowpass : TransferFcn  Numerator=1  Denominator=[sensor_noise_tau_position 1]
  X_White_Noise : RandomNumber  Variance=sigma_x^2  Seed=seed_x  SampleTime=sensor_sample_time
  Y_Measurement : Sum
  Y_Noise_Enable : Gain  Gain=sensor_noise_enabled
  Y_Noise_Lowpass : TransferFcn  Numerator=1  Denominator=[sensor_noise_tau_position 1]
  Y_White_Noise : RandomNumber  Variance=sigma_y^2  Seed=seed_y  SampleTime=sensor_sample_time
  Yaw_Measurement : Sum
  Yaw_Noise_Enable : Gain  Gain=sensor_noise_enabled
  Yaw_Noise_Lowpass : TransferFcn  Numerator=1  Denominator=[sensor_noise_tau_attitude 1]
  Yaw_White_Noise : RandomNumber  Variance=sigma_psi^2  Seed=seed_psi  SampleTime=sensor_sample_time
  Z_Measurement : Sum
  Z_Noise_Enable : Gain  Gain=sensor_noise_enabled
  Z_Noise_Lowpass : TransferFcn  Numerator=1  Denominator=[sensor_noise_tau_position 1]
  Z_White_Noise : RandomNumber  Variance=sigma_z^2  Seed=seed_z  SampleTime=sensor_sample_time
  x_meas : Outport
  y_meas : Outport  Port=2
  z_meas : Outport  Port=3
  phi_meas : Outport  Port=4
  theta_meas : Outport  Port=5
  psi_meas : Outport  Port=6
  wires:
  Yaw_Noise_Lowpass/1 -> Yaw_Noise_Enable/1
  Pitch_Noise_Lowpass/1 -> Pitch_Noise_Enable/1
  Roll_Noise_Lowpass/1 -> Roll_Noise_Enable/1
  Z_Noise_Lowpass/1 -> Z_Noise_Enable/1
  Y_Noise_Lowpass/1 -> Y_Noise_Enable/1
  X_Noise_Lowpass/1 -> X_Noise_Enable/1
  X_White_Noise/1 -> X_Noise_Lowpass/1
  x_true/1 -> X_Measurement/1
  X_Noise_Enable/1 -> X_Measurement/2
  X_Measurement/1 -> x_meas/1
  Y_White_Noise/1 -> Y_Noise_Lowpass/1
  y_true/1 -> Y_Measurement/1
  Y_Noise_Enable/1 -> Y_Measurement/2
  Y_Measurement/1 -> y_meas/1
  Z_White_Noise/1 -> Z_Noise_Lowpass/1
  z_true/1 -> Z_Measurement/1
  Z_Noise_Enable/1 -> Z_Measurement/2
  Z_Measurement/1 -> z_meas/1
  Roll_White_Noise/1 -> Roll_Noise_Lowpass/1
  phi_true/1 -> Roll_Measurement/1
  Roll_Noise_Enable/1 -> Roll_Measurement/2
  Roll_Measurement/1 -> phi_meas/1
  Pitch_White_Noise/1 -> Pitch_Noise_Lowpass/1
  theta_true/1 -> Pitch_Measurement/1
  Pitch_Noise_Enable/1 -> Pitch_Measurement/2
  Pitch_Measurement/1 -> theta_meas/1
  Yaw_White_Noise/1 -> Yaw_Noise_Lowpass/1
  psi_true/1 -> Yaw_Measurement/1
  Yaw_Noise_Enable/1 -> Yaw_Measurement/2
  Yaw_Measurement/1 -> psi_meas/1

== system Drone_Response_v5/Visualization_Output ==
  x_true : Inport
  y_true : Inport  Port=2
  z_true : Inport  Port=3
  phi_true : Inport  Port=4
  theta_true : Inport  Port=5
  psi_true : Inport  Port=6
  Flight_Visualization_Data : ToWorkspace  VariableName=flight_visualization  SaveFormat=Timeseries  SampleTime=-1
  State_Vector : Mux  Inputs=6
  wires:
  State_Vector/1 -> Flight_Visualization_Data/1  "state_3d"
  psi_true/1 -> State_Vector/6
  theta_true/1 -> State_Vector/5
  phi_true/1 -> State_Vector/4
  z_true/1 -> State_Vector/3
  y_true/1 -> State_Vector/2
  x_true/1 -> State_Vector/1

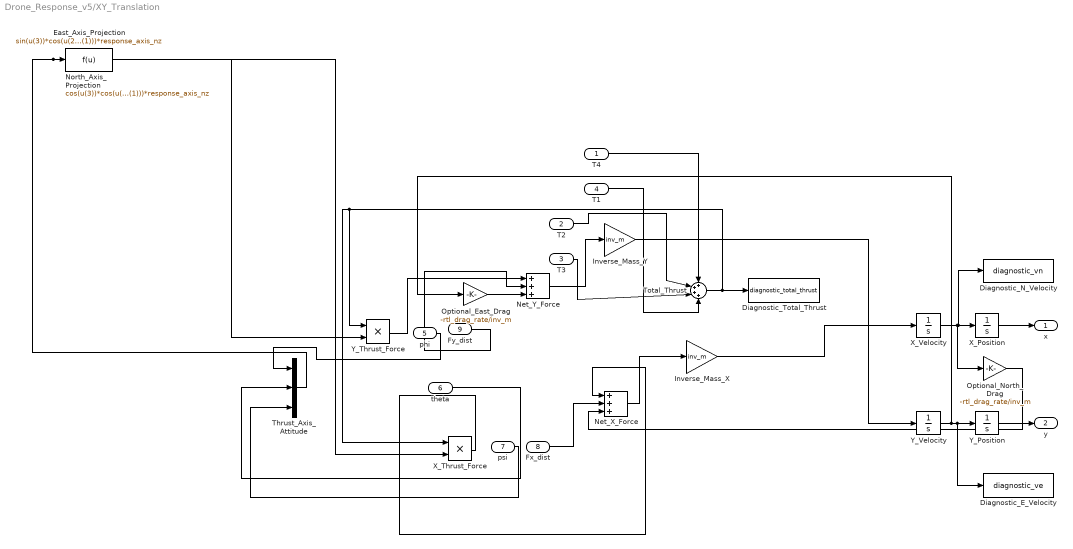
== system Drone_Response_v5/XY_Translation ==
  T4 : Inport
  T2 : Inport  Port=2
  T3 : Inport  Port=3
  T1 : Inport  Port=4
  phi : Inport  Port=5
  theta : Inport  Port=6
  psi : Inport  Port=7
  Fx_dist : Inport  Port=8
  Fy_dist : Inport  Port=9
  Diagnostic_E_Velocity : ToWorkspace  VariableName=diagnostic_ve  SaveFormat=Timeseries  SampleTime=-1
  Diagnostic_N_Velocity : ToWorkspace  VariableName=diagnostic_vn  SaveFormat=Timeseries  SampleTime=-1
  Diagnostic_Total_Thrust : ToWorkspace  VariableName=diagnostic_total_thrust  SaveFormat=Timeseries  SampleTime=-1
  East_Axis_Projection : Fcn  Expr=sin(u(3))*cos(u(2))*response_axis_nx+(sin(u(3))*sin(u(2))*sin(u(1))+cos(u(3))*cos(u(1)))*response_axis_ny+(sin(u(3))*sin(u(2))*cos(u(1))-cos(u(3))*sin(u(1)))*response_axis_nz
  Inverse_Mass_X : Gain  Gain=inv_m
  Inverse_Mass_Y : Gain  Gain=inv_m
  Net_X_Force : Sum  Inputs=+++
  Net_Y_Force : Sum  Inputs=+++
  North_Axis_Projection : Fcn  Expr=cos(u(3))*cos(u(2))*response_axis_nx+(cos(u(3))*sin(u(2))*sin(u(1))-sin(u(3))*cos(u(1)))*response_axis_ny+(cos(u(3))*sin(u(2))*cos(u(1))+sin(u(3))*sin(u(1)))*response_axis_nz
  Optional_East_Drag : Gain  Gain=-rtl_drag_rate/inv_m
  Optional_North_Drag : Gain  Gain=-rtl_drag_rate/inv_m
  Thrust_Axis_Attitude : Mux  Inputs=3
  Total_Thrust : Sum  Inputs=++++
  X_Position : Integrator  InitialCondition=x0
  X_Thrust_Force : Product
  X_Velocity : Integrator  InitialCondition=vx0
  Y_Position : Integrator  InitialCondition=y0
  Y_Thrust_Force : Product
  Y_Velocity : Integrator  InitialCondition=vy0
  x : Outport
  y : Outport  Port=2
  wires:
  X_Position/1 -> x/1
  T4/1 -> Total_Thrust/1
  Y_Position/1 -> y/1
  T1/1 -> Total_Thrust/4
  Net_X_Force/1 -> Inverse_Mass_X/1
  Fx_dist/1 -> Net_X_Force/2
  X_Thrust_Force/1 -> Net_X_Force/1
  Inverse_Mass_X/1 -> X_Velocity/1
  T2/1 -> Total_Thrust/2
  Inverse_Mass_Y/1 -> Y_Velocity/1
  T3/1 -> Total_Thrust/3
  Total_Thrust/1 -> Y_Thrust_Force/1, X_Thrust_Force/1, Diagnostic_Total_Thrust/1
  Optional_East_Drag/1 -> Net_Y_Force/3
  Optional_North_Drag/1 -> Net_X_Force/3
  X_Velocity/1 -> X_Position/1, Diagnostic_N_Velocity/1, Optional_North_Drag/1
  Y_Velocity/1 -> Y_Position/1, Diagnostic_E_Velocity/1, Optional_East_Drag/1
  Y_Thrust_Force/1 -> Net_Y_Force/1
  Fy_dist/1 -> Net_Y_Force/2
  Net_Y_Force/1 -> Inverse_Mass_Y/1
  phi/1 -> Thrust_Axis_Attitude/1
  theta/1 -> Thrust_Axis_Attitude/2
  psi/1 -> Thrust_Axis_Attitude/3
  Thrust_Axis_Attitude/1 -> East_Axis_Projection/1, North_Axis_Projection/1
  North_Axis_Projection/1 -> X_Thrust_Force/2
  East_Axis_Projection/1 -> Y_Thrust_Force/2
